simulink model "SimulinkAdsTest"  (R2020b)
(part 2 of 2)

      | 				<Text><![CDATA[InterpolationMode_Previous]]></Text>
      | 				<Enum>1</Enum>
      | 				<Comment><![CDATA[Take previous sample point]]></Comment>
      | 			</EnumInfo>
      | 			<EnumInfo>
      | 				<Text><![CDATA[InterpolationMode_Next]]></Text>
      | 				<Enum>2</Enum>
      | 				<Comment><![CDATA[Take following sample point]]></Comment>
      | 			</EnumInfo>
      | 			<EnumInfo>
      | 				<Text><![CDATA[InterpolationMode_Nearest]]></Text>
      | 				<Enum>3</Enum>
      | 				<Comment><![CDATA[Take nearest sample point]]></Comment>
      | 			</EnumInfo>
      | 			<EnumInfo>
      | 				<Text><![CDATA[InterpolationMode_Linear]]></Text>
      | 				<Enum>4</Enum>
      | 				<Comment><![CDATA[Linear interpolation]]></Comment>
      | 			</EnumInfo>
      | 			<Default>
      | 				<EnumText>InterpolationMode_Nearest</EnumText>
      | 			</Default>
      | 			<Hides>
      | 				<Hide GUID="{D1CE9774-5ABF-42E5-8FE4-99F5DEE76F36}"/>
      | 				<Hide GUID="{430DDA91-6797-4E3C-84C6-A1786F8B6EA7}"/>
      | 				<Hide GUID="{24DF4C47-A5FC-4534-A4AA-304CE11CAE9A}"/>
      | 				<Hide GUID="{5367B9B1-3807-4AFC-B79A-823BBFC694FE}"/>
      | 				<Hide GUID="{36E48A81-1480-4106-A31F-8CC0D9BDE1C1}"/>
      | 				<Hide GUID="{DB809631-0BE7-4AE2-8A30-534C3D3B8C19}"/>
      | 				<Hide GUID="{139A7071-B2F7-4999-AD00-5D72B7A47D1B}"/>
      | 				<Hide GUID="{E828C0A6-3D7C-424C-B6C8-3B4EEF9C18AC}"/>
      | 			</Hides>
      | 		</DataType>
      | 		<DataType>
      | 			<Name GUID="{B2873DF7-0E9A-4371-8FDA-560A407550FC}" Namespace="TcDataExchange">BufferReadExtrapolationMode</Name>
      | 			<BitSize>16</BitSize>
      | 			<BaseType GUID="{18071995-0000-0000-0000-000000000006}">INT</BaseType>
      | 			<EnumInfo>
      | 				<Text><![CDATA[ExtrapolationMode_None]]></Text>
      | 				<Enum>0</Enum>
      | 				<Comment><![CDATA[Return error, if the timestamp is out of the specified range]]></Comment>
      | 			</EnumInfo>
      | 			<EnumInfo>
      | 				<Text><![CDATA[ExtrapolationMode_Constant]]></Text>
      | 				<Enum>1</Enum>
      | 				<Comment><![CDATA[Use nearest sample point, if timestamp is out of the specified range]]></Comment>
      | 			</EnumInfo>
      | 			<EnumInfo>
      | 				<Text><![CDATA[ExtrapolationMode_Linear]]></Text>
      | 				<Enum>2</Enum>
      | 				<Comment><![CDATA[Extrapolate linearly, if timestamp is out of the specified range]]></Comment>
      | 			</EnumInfo>
      | 			<Hides>
      | 				<Hide GUID="{183AB6B0-9D13-4268-9013-6BC144AF43F9}"/>
      | 				<Hide GUID="{58686C98-6145-45BB-A1CE-6DFAFC306DB4}"/>
      | 				<Hide GUID="{EE21BE7C-9D24-4A92-825B-B15B1919983F}"/>
      | 				<Hide GUID="{98B9A1F3-AFB0-4DDD-856E-5CCA2E73CE75}"/>
      | 				<Hide GUID="{34806592-F19E-4DDB-96DC-032ABE8197D4}"/>
      | 				<Hide GUID="{C9391145-9682-4F6A-BF6D-5FA0733C02F4}"/>
      | 				<Hide GUID="{583534AC-9A1B-48FF-99BF-216BF02010E2}"/>
      | 				<Hide GUID="{11A9C8C7-1BFF-45E1-8ABC-29E82EA5F980}"/>
      | 				<Hide GUID="{CA042772-0740-496A-85A1-AE2E06F7EE08}"/>
      | 				<Hide GUID="{7F398EF7-03C7-49DC-B4A8-778E9B813ED0}"/>
      | 				<Hide GUID="{3075835C-D37D-4F7C-8CFA-0A55974D5F50}"/>
      | 			</Hides>
      | 		</DataType>
      | 		<DataType>
      | 			<Name GUID="{D7B34C9A-90C5-4E79-A290-017678319005}" Namespace="TcDataExchange">ITcStreamAdsRequestHandler</Name>
      | 			<BitSize X64="64">32</BitSize>
      | 			<BaseType GUID="{00000001-0000-0000-E000-000000000064}">ITcUnknown</BaseType>
      | 			<Method>
      | 				<Name>Send</Name>
      | 				<ReturnType GUID="{18071995-0000-0000-0000-000000000019}">HRESULT</ReturnType>
      | 				<ReturnBitSize>32</ReturnBitSize>
      | 				<Parameter>
      | 					<Name>timeoutMs</Name>
      | 					<Type GUID="{18071995-0000-0000-0000-000000000006}" Optional="1000">INT</Type>
      | 					<BitSize>16</BitSize>
      | 				</Parameter>
      | 			</Method>
      | 			<Method>
      | 				<Name>GetResult</Name>
      | 				<ReturnType GUID="{18071995-0000-0000-0000-000000000019}">HRESULT</ReturnType>
      | 				<ReturnBitSize>32</ReturnBitSize>
      | 				<Parameter>
      | 					<Name>pErrorCode</Name>
      | 					<Type GUID="{18071995-0000-0000-0000-000000000009}" PointerTo="1" RpcDirection="out">DINT</Type>
      | 					<BitSize X64="64">32</BitSize>
      | 				</Parameter>
      | 				<Parameter>
      | 					<Name>wait</Name>
      | 					<Type GUID="{18071995-0000-0000-0000-000000000030}" Optional="0">BOOL</Type>
      | 					<BitSize>8</BitSize>
      | 				</Parameter>
      | 			</Method>
      | 			<Method>
      | 				<Name>Cancel</Name>
      | 				<ReturnType GUID="{18071995-0000-0000-0000-000000000019}">HRESULT</ReturnType>
      | 				<ReturnBitSize>32</ReturnBitSize>
      | 			</Method>
      | 			<Hides>
      | 				<Hide GUID="{D5D4EABE-5709-4F1D-A52D-DD780CF3BEE8}"/>
      | 				<Hide GUID="{96230612-048D-4927-9A3E-E69B743416F7}"/>
      | 				<Hide GUID="{F0F623C7-A650-457C-A27C-87DC2B08989E}"/>
      | 				<Hide GUID="{18FCA6B6-AFA6-45DD-BC02-F3037EA03FB7}"/>
      | 				<Hide GUID="{12AC5FFF-B3F6-4F3E-8EDD-8044D44F084F}"/>
      | 				<Hide GUID="{6CDF8435-1307-4137-94DE-D793A77839C3}"/>
      | 			</Hides>
      | 		</DataType>
      | 		<DataType>
      | 			<Name GUID="{18071995-0000-0000-0000-000000000041}" TcBaseType="true" HideSubItems="true" CName="AmsNetId">AMSNETID</Name>
      | 			<BitSize>48</BitSize>
      | 			<BaseType GUID="{18071995-0000-0000-0000-000000000001}">BYTE</BaseType>
      | 			<ArrayInfo>
      | 				<LBound>0</LBound>
      | 				<Elements>6</Elements>
      | 			</ArrayInfo>
      | 			<Format>
      | 				<Printf>%d.%d.%d.%d.%d.%d</Printf>
      | 				<Parameter>[0]</Parameter>
      | 				<Parameter>[1]</Parameter>
      | 				<Parameter>[2]</Parameter>
      | 				<Parameter>[3]</Parameter>
      | 				<Parameter>[4]</Parameter>
      | 				<Parameter>[5]</Parameter>
      | 			</Format>
      | 		</DataType>
      | 		<DataType>
      | 			<Name GUID="{18071995-0000-0000-0000-000000000042}" TcBaseType="true" CName="AmsAddr">AMSADDR</Name>
      | 			<BitSize>64</BitSize>
      | 			<SubItem>
      | 				<Name>netId</Name>
      | 				<Type GUID="{18071995-0000-0000-0000-000000000041}">AMSNETID</Type>
      | 				<BitSize>48</BitSize>
      | 				<BitOffs>0</BitOffs>
      | 			</SubItem>
      | 			<SubItem>
      | 				<Name>port</Name>
      | 				<Type GUID="{18071995-0000-0000-0000-000000000004}">WORD</Type>
      | 				<BitSize>16</BitSize>
      | 				<BitOffs>48</BitOffs>
      | 			</SubItem>
      | 			<Format>
      | 				<Printf>%d.%d.%d.%d.%d.%d:%d</Printf>
      | 				<Parameter>.netId[0]</Parameter>
      | 				<Parameter>.netId[1]</Parameter>
      | 				<Parameter>.netId[2]</Parameter>
      | 				<Parameter>.netId[3]</Parameter>
      | 				<Parameter>.netId[4]</Parameter>
      | 				<Parameter>.netId[5]</Parameter>
      | 				<Parameter>.port</Parameter>
      | 			</Format>
      | 			<Format Name="Iec">
      | 				<Printf>(netId:=[%d.%d.%d.%d.%d.%d], port :=%d)</Printf>
      | 				<Parameter>.netId[0]</Parameter>
      | 				<Parameter>.netId[1]</Parameter>
      | 				<Parameter>.netId[2]</Parameter>
      | 				<Parameter>.netId[3]</Parameter>
      | 				<Parameter>.netId[4]</Parameter>
      | 				<Parameter>.netId[5]</Parameter>
      | 				<Parameter>.port</Parameter>
      | 			</Format>
      | 		</DataType>
      | 		<DataType>
      | 			<Name GUID="{2919D6B4-47C4-4AE8-B706-E94C497ECB99}" Namespace="TcDataExchange">NotificationTransMode</Name>
      | 			<BitSize>16</BitSize>
      | 			<BaseType GUID="{18071995-0000-0000-0000-000000000006}">INT</BaseType>
      | 			<EnumInfo>
      | 				<Text><![CDATA[NoTrans]]></Text>
      | 				<Enum>0</Enum>
      | 			</EnumInfo>
      | 			<EnumInfo>
      | 				<Text><![CDATA[ServerCycle]]></Text>
      | 				<Enum>3</Enum>
      | 			</EnumInfo>
      | 			<EnumInfo>
      | 				<Text><![CDATA[OnChange]]></Text>
      | 				<Enum>4</Enum>
      | 			</EnumInfo>
      | 			<Hides>
      | 				<Hide GUID="{79465139-46B4-43EB-B7FF-967BF64C3367}"/>
      | 				<Hide GUID="{AE2F4BB5-B98E-4C79-AC26-086A9CF7EAC6}"/>
      | 				<Hide GUID="{ECF929B2-79C7-483F-A3DC-06B91AFD531C}"/>
      | 				<Hide GUID="{4E4B27B2-E550-42F1-92B6-1EFABDB0481B}"/>
      | 			</Hides>
      | 		</DataType>
      | 		<DataType>
      | 			<Name GUID="{B75DDCED-7BC8-45F5-8D80-27345642612D}" Namespace="TcDataExchange">NotificationState</Name>
      | 			<BitSize>16</BitSize>
      | 			<BaseType GUID="{18071995-0000-0000-0000-000000000006}">INT</BaseType>
      | 			<EnumInfo>
      | 				<Text><![CDATA[Stop]]></Text>
      | 				<Enum>0</Enum>
      | 			</EnumInfo>
      | 			<EnumInfo>
      | 				<Text><![CDATA[Starting]]></Text>
      | 				<Enum>1</Enum>
      | 			</EnumInfo>
      | 			<EnumInfo>
      | 				<Text><![CDATA[Run]]></Text>
      | 				<Enum>2</Enum>
      | 			</EnumInfo>
      | 			<EnumInfo>
      | 				<Text><![CDATA[Stopping]]></Text>
      | 				<Enum>3</Enum>
      | 			</EnumInfo>
      | 			<EnumInfo>
      | 				<Text><![CDATA[StartError]]></Text>
      | 				<Enum>4</Enum>
      | 			</EnumInfo>
      | 			<EnumInfo>
      | 				<Text><![CDATA[StopError]]></Text>
      | 				<Enum>5</Enum>
      | 			</EnumInfo>
      | 			<Hides>
      | 				<Hide GUID="{BEEA3766-C152-4B4D-80E7-6332297C102B}"/>
      | 			</Hides>
      | 		</DataType>
      | 		<DataType>
      | 			<Name GUID="{7BD2CA64-894F-4710-AF21-189254BD7339}" Namespace="TcDataExchange">ITcStreamAdsNotificationHandler</Name>
      | 			<BitSize X64="64">32</BitSize>
      | 			<BaseType GUID="{00000001-0000-0000-E000-000000000064}">ITcUnknown</BaseType>
      | 			<Method>
      | 				<Name>Start</Name>
      | 				<ReturnType GUID="{18071995-0000-0000-0000-000000000019}">HRESULT</ReturnType>
      | 				<ReturnBitSize>32</ReturnBitSize>
      | 				<Parameter>
      | 					<Name>sampleTime100ns</Name>
      | 					<Comment><![CDATA[SampleTime in 100ns. If the value is 0 or too small, the requests will be send as fast as possible.]]></Comment>
      | 					<Type GUID="{18071995-0000-0000-0000-000000000008}" Optional="0">UDINT</Type>
      | 					<BitSize>32</BitSize>
      | 				</Parameter>
      | 				<Parameter>
      | 					<Name>delayTime100ns</Name>
      | 					<Comment><![CDATA[DelayTime in 100ns.]]></Comment>
      | 					<Type GUID="{18071995-0000-0000-0000-000000000008}" Optional="10">UDINT</Type>
      | 					<BitSize>32</BitSize>
      | 				</Parameter>
      | 				<Parameter>
      | 					<Name>createTimeoutMs</Name>
      | 					<Type GUID="{18071995-0000-0000-0000-000000000006}" Optional="1000">INT</Type>
      | 					<BitSize>16</BitSize>
      | 				</Parameter>
      | 				<Parameter>
      | 					<Name>transMode</Name>
      | 					<Type GUID="{2919D6B4-47C4-4AE8-B706-E94C497ECB99}" Namespace="TcDataExchange" Optional="0">NotificationTransMode</Type>
      | 					<BitSize>16</BitSize>
      | 				</Parameter>
      | 			</Method>
      | 			<Method>
      | 				<Name>Stop</Name>
      | 				<ReturnType GUID="{18071995-0000-0000-0000-000000000019}">HRESULT</ReturnType>
      | 				<ReturnBitSize>32</ReturnBitSize>
      | 				<Parameter>
      | 					<Name>stopTimeoutMs</Name>
      | 					<Type GUID="{18071995-0000-0000-0000-000000000006}" Optional="1000">INT</Type>
      | 					<BitSize>16</BitSize>
      | 				</Parameter>
      | 			</Method>
      | 			<Method>
      | 				<Name>GetState</Name>
      | 				<ReturnType GUID="{18071995-0000-0000-0000-000000000019}">HRESULT</ReturnType>
      | 				<ReturnBitSize>32</ReturnBitSize>
      | 				<Parameter>
      | 					<Name>pState</Name>
      | 					<Type GUID="{B75DDCED-7BC8-45F5-8D80-27345642612D}" Namespace="TcDataExchange" PointerTo="1">NotificationState</Type>
      | 					<BitSize X64="64">32</BitSize>
      | 				</Parameter>
      | 				<Parameter>
      | 					<Name>pErrorCode</Name>
      | 					<Type GUID="{18071995-0000-0000-0000-000000000009}" PointerTo="1">DINT</Type>
      | 					<BitSize X64="64">32</BitSize>
      | 				</Parameter>
      | 			</Method>
      | 			<Method>
      | 				<Name>WaitFor</Name>
      | 				<ReturnType GUID="{18071995-0000-0000-0000-000000000019}">HRESULT</ReturnType>
      | 				<ReturnBitSize>32</ReturnBitSize>
      | 				<Parameter>
      | 					<Name>targetState</Name>
      | 					<Type GUID="{B75DDCED-7BC8-45F5-8D80-27345642612D}" Namespace="TcDataExchange">NotificationState</Type>
      | 					<BitSize>16</BitSize>
      | 				</Parameter>
      | 			</Method>
      | 			<Hides>
      | 				<Hide GUID="{0FD54C3A-649C-4819-BA34-40090DB2854F}"/>
      | 				<Hide GUID="{B851627D-4078-4428-873B-9E0DE756697F}"/>
      | 				<Hide GUID="{82738EA0-63AE-4386-9AC8-D5A166BE7CE6}"/>
      | 				<Hide GUID="{62C58600-337E-4913-B519-B241B47A093F}"/>
      | 				<Hide GUID="{F19E62E1-3672-44A5-AE6F-41D70903D13E}"/>
      | 				<Hide GUID="{188DFF90-A46E-4A6C-BF2A-4B79F1A4A7D7}"/>
      | 				<Hide GUID="{20D7666F-EA21-4A02-B0BF-92A2B39D0282}"/>
      | 				<Hide GUID="{B6680295-EE8B-49D4-B982-46287CB9DC7F}"/>
      | 				<Hide GUID="{640F79DB-CF38-45B7-A5A6-1F8ACF6E88C7}"/>
      | 				<Hide GUID="{ACD4E2BC-BCCF-47C3-994A-79C84DA897B4}"/>
      | 			</Hides>
      | 		</DataType>
      | 		<DataType>
      | 			<Name GUID="{44CF19E6-1A23-4E07-B15E-18C86B7D1DF6}" Namespace="TcDataExchange">ITcStreamAdsClient</Name>
      | 			<BitSize X64="64">32</BitSize>
      | 			<BaseType GUID="{00000001-0000-0000-E000-000000000064}">ITcUnknown</BaseType>
      | 			<Method>
      | 				<Name>CreateReadRequest</Name>
      | 				<ReturnType GUID="{18071995-0000-0000-0000-000000000019}">HRESULT</ReturnType>
      | 				<ReturnBitSize>32</ReturnBitSize>
      | 				<Parameter>
      | 					<Name>parentOid</Name>
      | 					<Type GUID="{18071995-0000-0000-0000-00000000000F}">OTCID</Type>
      | 					<BitSize>32</BitSize>
      | 				</Parameter>
      | 				<Parameter>
      | 					<Name>ppRequestHandler</Name>
      | 					<Type GUID="{D7B34C9A-90C5-4E79-A290-017678319005}" Namespace="TcDataExchange" PointerTo="1" RpcDirection="out">ITcStreamAdsRequestHandler</Type>
      | 					<BitSize X64="64">32</BitSize>
      | 				</Parameter>
      | 				<Parameter>
      | 					<Name>amsAddr</Name>
      | 					<Type GUID="{18071995-0000-0000-0000-000000000042}" RpcDirection="in">AMSADDR</Type>
      | 					<BitSize>64</BitSize>
      | 				</Parameter>
      | 				<Parameter>
      | 					<Name>idxGrp</Name>
      | 					<Type GUID="{18071995-0000-0000-0000-000000000008}" RpcDirection="in">UDINT</Type>
      | 					<BitSize>32</BitSize>
      | 				</Parameter>
      | 				<Parameter>
      | 					<Name>idxOffs</Name>
      | 					<Type GUID="{18071995-0000-0000-0000-000000000008}" RpcDirection="in">UDINT</Type>
      | 					<BitSize>32</BitSize>
      | 				</Parameter>
      | 				<Parameter>
      | 					<Name>byteSize</Name>
      | 					<Type GUID="{18071995-0000-0000-0000-000000000008}" RpcDirection="in">UDINT</Type>
      | 					<BitSize>32</BitSize>
      | 				</Parameter>
      | 				<Parameter>
      | 					<Name>pSink</Name>
      | 					<Type GUID="{CD026BE9-DD1E-4238-B09F-CDE426934EFB}" Namespace="TcDataExchange" RpcDirection="in">ITcStreamSyncDataSink</Type>
      | 					<BitSize X64="64">32</BitSize>
      | 				</Parameter>
      | 			</Method>
      | 			<Method>
      | 				<Name>CreateWriteRequest</Name>
      | 				<ReturnType GUID="{18071995-0000-0000-0000-000000000019}">HRESULT</ReturnType>
      | 				<ReturnBitSize>32</ReturnBitSize>
      | 				<Parameter>
      | 					<Name>parentOid</Name>
      | 					<Type GUID="{18071995-0000-0000-0000-00000000000F}">OTCID</Type>
      | 					<BitSize>32</BitSize>
      | 				</Parameter>
      | 				<Parameter>
      | 					<Name>ppRequestHandler</Name>
      | 					<Type GUID="{D7B34C9A-90C5-4E79-A290-017678319005}" Namespace="TcDataExchange" PointerTo="1" RpcDirection="out">ITcStreamAdsRequestHandler</Type>
      | 					<BitSize X64="64">32</BitSize>
      | 				</Parameter>
      | 				<Parameter>
      | 					<Name>amsAddr</Name>
      | 					<Type GUID="{18071995-0000-0000-0000-000000000042}" RpcDirection="in">AMSADDR</Type>
      | 					<BitSize>64</BitSize>
      | 				</Parameter>
      | 				<Parameter>
      | 					<Name>idxGrp</Name>
      | 					<Type GUID="{18071995-0000-0000-0000-000000000008}" RpcDirection="in">UDINT</Type>
      | 					<BitSize>32</BitSize>
      | 				</Parameter>
      | 				<Parameter>
      | 					<Name>idxOffs</Name>
      | 					<Type GUID="{18071995-0000-0000-0000-000000000008}" RpcDirection="in">UDINT</Type>
      | 					<BitSize>32</BitSize>
      | 				</Parameter>
      | 				<Parameter>
      | 					<Name>byteSize</Name>
      | 					<Type GUID="{18071995-0000-0000-0000-000000000008}" RpcDirection="in">UDINT</Type>
      | 					<BitSize>32</BitSize>
      | 				</Parameter>
      | 				<Parameter>
      | 					<Name>pSource</Name>
      | 					<Type GUID="{877CB26F-4EC1-469B-9F87-706DDBDA821F}" Namespace="TcDataExchange" RpcDirection="in">ITcStreamSyncDataSource</Type>
      | 					<BitSize X64="64">32</BitSize>
      | 				</Parameter>
      | 			</Method>
      | 			<Method>
      | 				<Name>CreateReadWriteRequest</Name>
      | 				<ReturnType GUID="{18071995-0000-0000-0000-000000000019}">HRESULT</ReturnType>
      | 				<ReturnBitSize>32</ReturnBitSize>
      | 				<Parameter>
      | 					<Name>parentOid</Name>
      | 					<Type GUID="{18071995-0000-0000-0000-00000000000F}">OTCID</Type>
      | 					<BitSize>32</BitSize>
      | 				</Parameter>
      | 				<Parameter>
      | 					<Name>ppRequestHandler</Name>
      | 					<Type GUID="{D7B34C9A-90C5-4E79-A290-017678319005}" Namespace="TcDataExchange" PointerTo="1" RpcDirection="out">ITcStreamAdsRequestHandler</Type>
      | 					<BitSize X64="64">32</BitSize>
      | 				</Parameter>
      | 				<Parameter>
      | 					<Name>amsAddr</Name>
      | 					<Type GUID="{18071995-0000-0000-0000-000000000042}" RpcDirection="in">AMSADDR</Type>
      | 					<BitSize>64</BitSize>
      | 				</Parameter>
      | 				<Parameter>
      | 					<Name>idxGrp</Name>
      | 					<Type GUID="{18071995-0000-0000-0000-000000000008}" RpcDirection="in">UDINT</Type>
      | 					<BitSize>32</BitSize>
      | 				</Parameter>
      | 				<Parameter>
      | 					<Name>idxOffs</Name>
      | 					<Type GUID="{18071995-0000-0000-0000-000000000008}" RpcDirection="in">UDINT</Type>
      | 					<BitSize>32</BitSize>
      | 				</Parameter>
      | 				<Parameter>
      | 					<Name>writeSize</Name>
      | 					<Type GUID="{18071995-0000-0000-0000-000000000008}" RpcDirection="in">UDINT</Type>
      | 					<BitSize>32</BitSize>
      | 				</Parameter>
      | 				<Parameter>
      | 					<Name>pSource</Name>
      | 					<Type GUID="{877CB26F-4EC1-469B-9F87-706DDBDA821F}" Namespace="TcDataExchange" RpcDirection="in">ITcStreamSyncDataSource</Type>
      | 					<BitSize X64="64">32</BitSize>
      | 				</Parameter>
      | 				<Parameter>
      | 					<Name>readSize</Name>
      | 					<Type GUID="{18071995-0000-0000-0000-000000000008}" RpcDirection="in">UDINT</Type>
      | 					<BitSize>32</BitSize>
      | 				</Parameter>
      | 				<Parameter>
      | 					<Name>pSink</Name>
      | 					<Type GUID="{CD026BE9-DD1E-4238-B09F-CDE426934EFB}" Namespace="TcDataExchange" RpcDirection="in">ITcStreamSyncDataSink</Type>
      | 					<BitSize X64="64">32</BitSize>
      | 				</Parameter>
      | 			</Method>
      | 			<Method>
      | 				<Name>CreateNotificationHandler</Name>
      | 				<ReturnType GUID="{18071995-0000-0000-0000-000000000019}">HRESULT</ReturnType>
      | 				<ReturnBitSize>32</ReturnBitSize>
      | 				<Parameter>
      | 					<Name>parentOid</Name>
      | 					<Type GUID="{18071995-0000-0000-0000-00000000000F}">OTCID</Type>
      | 					<BitSize>32</BitSize>
      | 				</Parameter>
      | 				<Parameter>
      | 					<Name>ppNotificationHandler</Name>
      | 					<Type GUID="{7BD2CA64-894F-4710-AF21-189254BD7339}" Namespace="TcDataExchange" PointerTo="1" RpcDirection="out">ITcStreamAdsNotificationHandler</Type>
      | 					<BitSize X64="64">32</BitSize>
      | 				</Parameter>
      | 				<Parameter>
      | 					<Name>amsAddr</Name>
      | 					<Type GUID="{18071995-0000-0000-0000-000000000042}">AMSADDR</Type>
      | 					<BitSize>64</BitSize>
      | 				</Parameter>
      | 				<Parameter>
      | 					<Name>idxGrp</Name>
      | 					<Type GUID="{18071995-0000-0000-0000-000000000008}" RpcDirection="in">UDINT</Type>
      | 					<BitSize>32</BitSize>
      | 				</Parameter>
      | 				<Parameter>
      | 					<Name>idxOffs</Name>
      | 					<Type GUID="{18071995-0000-0000-0000-000000000008}" RpcDirection="in">UDINT</Type>
      | 					<BitSize>32</BitSize>
      | 				</Parameter>
      | 				<Parameter>
      | 					<Name>byteSize</Name>
      | 					<Type GUID="{18071995-0000-0000-0000-000000000008}" RpcDirection="in">UDINT</Type>
      | 					<BitSize>32</BitSize>
      | 				</Parameter>
      | 				<Parameter>
      | 					<Name>pSink</Name>
      | 					<Type GUID="{CD026BE9-DD1E-4238-B09F-CDE426934EFB}" Namespace="TcDataExchange" RpcDirection="in">ITcStreamSyncDataSink</Type>
      | 					<BitSize X64="64">32</BitSize>
      | 				</Parameter>
      | 			</Method>
      | 			<Hides>
      | 				<Hide GUID="{E5572F78-39F4-4573-890C-3DF0E2006105}"/>
      | 				<Hide GUID="{52252529-8C17-45D1-85B4-6A458C0F3E94}"/>
      | 				<Hide GUID="{F824C7E1-F0C6-44A6-B482-897B83EFF54D}"/>
      | 				<Hide GUID="{89D1DEF9-1EDB-4DC7-B44F-67745448E326}"/>
      | 				<Hide GUID="{9AF2891A-A1C3-41B4-843B-F1318836B90C}"/>
      | 				<Hide GUID="{C92F8EE8-70FC-4938-AE5D-0804054FE778}"/>
      | 				<Hide GUID="{692D2F91-2921-429B-A2FD-B23E2D06FE57}"/>
      | 				<Hide GUID="{247F4AE9-8FC4-4311-BF3B-2963D4FB048A}"/>
      | 				<Hide GUID="{FB8AA9BF-37B4-4992-B5AC-BBA0F4D43373}"/>
      | 				<Hide GUID="{7427C36F-E349-41A6-A066-CB0C042DD556}"/>
      | 				<Hide GUID="{E46C7F48-0073-45AF-850A-7F1CB9D0F1BC}"/>
      | 				<Hide GUID="{096DB961-B576-4662-AA01-00D308385BF0}"/>
      | 				<Hide GUID="{A0AD0C9E-66BD-49F7-B782-910B430A1CD8}"/>
      | 				<Hide GUID="{FA6AC3AF-43AA-44CB-BA36-5723B1AD464D}"/>
      | 				<Hide GUID="{0614F527-21B4-4192-AE03-7FDCC97AD564}"/>
      | 				<Hide GUID="{20F9385A-0313-4208-B227-DA4EACC1424F}"/>
      | 				<Hide GUID="{DBEA0444-99ED-4B99-9B51-31DB70AF46EF}"/>
      | 				<Hide GUID="{C3B2FC5E-7AD1-45D8-9723-AA6C61AD9B60}"/>
      | 				<Hide GUID="{CF97D717-7515-4E5A-BE1F-84F5A676B8F8}"/>
      | 				<Hide GUID="{B3BDED57-1312-4D96-B06F-2628ECBA6EEF}"/>
      | 				<Hide GUID="{5DE91436-84B1-4D76-B0CA-1D6620CA428C}"/>
      | 				<Hide GUID="{A0E457C6-B984-4427-829D-FA992FA6D9F8}"/>
      | 				<Hide GUID="{49669A99-FF7E-4056-9658-FDC96AB6BD99}"/>
      | 				<Hide GUID="{53867E37-5FD2-456B-BE41-4F337E21E47A}"/>
      | 				<Hide GUID="{A3973658-0AF9-4706-9520-0AAF0F575BFE}"/>
      | 				<Hide GUID="{FC062AA8-EE46-46C7-94CF-827603675385}"/>
      | 				<Hide GUID="{021F7DA4-A9B9-4EF5-80F9-A8DBC397B675}"/>
      | 				<Hide GUID="{4D5006B6-E8E6-4498-9498-ACA7E948FC8F}"/>
      | 				<Hide GUID="{984AB404-08AC-4281-AB66-6ED5B3F17DFE}"/>
      | 				<Hide GUID="{D581F6CF-93AC-4E4B-8D6F-3F0EF3492A71}"/>
      | 				<Hide GUID="{7A32D7B0-99BA-4055-815F-11160248ACD0}"/>
      | 				<Hide GUID="{9E7FC559-CAD5-43C8-B16B-2E56C1991573}"/>
      | 				<Hide GUID="{F062CF59-8FAE-4FCB-A01C-9B649900BCA5}"/>
      | 				<Hide GUID="{8728E0D9-0A46-4A30-9F10-DD1BF2EA33CE}"/>
      | 				<Hide GUID="{DFBB006E-343D-4910-A9C8-3AB2FE1535D3}"/>
      | 				<Hide GUID="{28C016BE-C467-4209-83F6-DED24711BF6D}"/>
      | 				<Hide GUID="{090DBC60-C9BC-4AB3-B82F-77F59E060169}"/>
      | 				<Hide GUID="{7C69CB05-063E-4BC5-9379-7224930A2D33}"/>
      | 				<Hide GUID="{AFAD7A5B-01FD-4391-87A6-15283DC78C95}"/>
      | 				<Hide GUID="{5E61A921-550A-4063-9429-A8A28DE5A1E3}"/>
      | 				<Hide GUID="{6BB012C3-FEAE-471E-BD95-27EDA5BB3A24}"/>
      | 				<Hide GUID="{E5B9394C-8543-4D1E-86CA-EC772D80F874}"/>
      | 				<Hide GUID="{B8FC3674-8C27-4962-8D53-5010B3276572}"/>
      | 				<Hide GUID="{7A879166-081C-4396-83F5-1ED6DDC3FE02}"/>
      | 				<Hide GUID="{906345FE-D08D-48EB-B8DC-3909739597CB}"/>
      | 			</Hides>
      | 		</DataType>
      | 	</DataTypes>
      | 	<Translations/>
      | 	<System>
      | 		<Tasks>
      | 			<Task ObjectId="33620000" CycleTime="100000" AmsPort="350" Priority="20">
      | 				<Name>TcDataExchangeModulesTask</Name>
      | 			</Task>
      | 		</Tasks>
      | 		<Modules>
      | 			<Module GUID="{AB7EF359-EC28-4A80-B6B9-1F5FEF806409}" ClassFactoryId="Beckhoff Automation|TcDataExchangeModules|1.0.1.166" Group="DataExchange|StreamUtilities">
      | 				<Name>Synchronizer</Name>
      | 				<CLSID ClassFactory="TcDataExchangeModules">{AB7EF359-EC28-4A80-B6B9-1F5FEF806409}</CLSID>
      | 				<Info/>
      | 				<Licenses>
      | 					<License>
      | 						<LicenseId>{304D006A-8299-4560-AB79-438534B50288}</LicenseId>
      | 					</License>
      | 				</Licenses>
      | 				<InitSequence>SO</InitSequence>
      | 				<Contexts>
      | 					<Context>
      | 						<Id>1</Id>
      | 					</Context>
      | 				</Contexts>
      | 				<Interfaces>
      | 					<Interface DisableCodeGeneration="true">
      | 						<Type GUID="{00000012-0000-0000-E000-000000000064}">ITComObject</Type>
      | 					</Interface>
      | 					<Interface DisableCodeGeneration="true">
      | 						<Type GUID="{03000012-0000-0000-E000-000000000064}">ITcADI</Type>
      | 					</Interface>
      | 					<Interface DisableCodeGeneration="true">
      | 						<Type GUID="{03000018-0000-0000-E000-000000000064}">ITcWatchSource</Type>
      | 					</Interface>
      | 					<Interface>
      | 						<Type GUID="{9165C8A1-78D1-4B81-89D0-BA48F61AF93B}" Namespace="TcDataExchange">ITcStreamSynchronizer</Type>
      | 					</Interface>
      | 				</Interfaces>
      | 				<Parameters>
      | 					<Parameter HideParameter="true">
      | 						<Name>TraceLevelMax</Name>
      | 						<Comment TxtId=""><![CDATA[Controls the amount of log messages.]]></Comment>
      | 						<BitSize>32</BitSize>
      | 						<BaseType GUID="{8007AE3B-86BB-40F2-B385-EF87FCC239A4}">TcTraceLevel</BaseType>
      | 						<PTCID>#x03002103</PTCID>
      | 						<ContextId>1</ContextId>
      | 					</Parameter>
      | 				</Parameters>
      | 				<InstanceName>Synchronizer_Instance1</InstanceName>
      | 				<OTCID>#x01010010</OTCID>
      | 				<ParameterValues>
      | 					<Value>
      | 						<Name>TraceLevelMax</Name>
      | 						<EnumText>tlAlways</EnumText>
      | 					</Value>
      | 				</ParameterValues>
      | 			</Module>
      | 			<Module GUID="{7F2917A9-6092-40A6-BB22-5428D680BA27}" ClassFactoryId="Beckhoff Automation|TcDataExchangeModules|1.0.1.166" Group="DataExchange|StreamUtilities">
      | 				<Name>SyncBuffer</Name>
      | 				<CLSID ClassFactory="TcDataExchangeModules">{7F2917A9-6092-40A6-BB22-5428D680BA27}</CLSID>
      | 				<Info/>
      | 				<Licenses>
      | 					<License>
      | 						<LicenseId>{304D006A-8299-4560-AB79-438534B50288}</LicenseId>
      | 					</License>
      | 				</Licenses>
      | 				<InitSequence>SO</InitSequence>
      | 				<Contexts>
      | 					<Context>
      | 						<Id>1</Id>
      | 					</Context>
      | 				</Contexts>
      | 				<Interfaces>
      | 					<Interface DisableCodeGeneration="true">
      | 						<Type GUID="{00000012-0000-0000-E000-000000000064}">ITComObject</Type>
      | 					</Interface>
      | 					<Interface DisableCodeGeneration="true">
      | 						<Type GUID="{03000012-0000-0000-E000-000000000064}">ITcADI</Type>
      | 					</Interface>
      | 					<Interface DisableCodeGeneration="true">
      | 						<Type GUID="{03000018-0000-0000-E000-000000000064}">ITcWatchSource</Type>
      | 					</Interface>
      | 					<Interface>
      | 						<Type GUID="{CD026BE9-DD1E-4238-B09F-CDE426934EFB}" Namespace="TcDataExchange">ITcStreamSyncDataSink</Type>
      | 					</Interface>
      | 					<Interface>
      | 						<Type GUID="{877CB26F-4EC1-469B-9F87-706DDBDA821F}" Namespace="TcDataExchange">ITcStreamSyncDataSource</Type>
      | 					</Interface>
      | 					<Interface>
      | 						<Type GUID="{CC2323D2-5F91-43AC-9820-54D42A9D0317}" Namespace="TcDataExchange">ITcStreamBuffer</Type>
      | 					</Interface>
      | 				</Interfaces>
      | 				<Parameters>
      | 					<Parameter>
      | 						<Name>InterpolationMode</Name>
      | 						<BitSize>16</BitSize>
      | 						<BaseType GUID="{04A85163-BBE2-45EF-A167-1FD20C2F2D46}" Namespace="TcDataExchange">BufferReadInterpolationMode</BaseType>
      | 						<PTCID>#x00000004</PTCID>
      | 						<ContextId>1</ContextId>
      | 					</Parameter>
      | 					<Parameter>
      | 						<Name>ContinuationMode</Name>
      | 						<BitSize>16</BitSize>
      | 						<BaseType GUID="{B2873DF7-0E9A-4371-8FDA-560A407550FC}" Namespace="TcDataExchange">BufferReadExtrapolationMode</BaseType>
      | 						<PTCID>#x00000005</PTCID>
      | 						<ContextId>1</ContextId>
      | 					</Parameter>
      | 					<Parameter>
      | 						<Name>SampleSize</Name>
      | 						<BitSize>32</BitSize>
      | 						<BaseType GUID="{18071995-0000-0000-0000-000000000008}">UDINT</BaseType>
      | 						<PTCID>#x00000006</PTCID>
      | 						<ContextId>1</ContextId>
      | 					</Parameter>
      | 					<Parameter>
      | 						<Name>Capacity</Name>
      | 						<BitSize>32</BitSize>
      | 						<BaseType GUID="{18071995-0000-0000-0000-000000000008}">UDINT</BaseType>
      | 						<PTCID>#x00000007</PTCID>
      | 						<ContextId>1</ContextId>
      | 					</Parameter>
      | 					<Parameter HideParameter="true">
      | 						<Name>TraceLevelMax</Name>
      | 						<Comment TxtId=""><![CDATA[Controls the amount of log messages.]]></Comment>
      | 						<BitSize>32</BitSize>
      | 						<BaseType GUID="{8007AE3B-86BB-40F2-B385-EF87FCC239A4}">TcTraceLevel</BaseType>
      | 						<PTCID>#x03002103</PTCID>
      | 						<ContextId>1</ContextId>
      | 					</Parameter>
      | 				</Parameters>
      | 				<InterfacePointers>
      | 					<InterfacePointer>
      | 						<PTCID>#x00000001</PTCID>
      | 						<Name>Synchronizer</Name>
      | 						<Type GUID="{9165C8A1-78D1-4B81-89D0-BA48F61AF93B}" Namespace="TcDataExchange">ITcStreamSynchronizer</Type>
      | 						<ContextId>1</ContextId>
      | 					</InterfacePointer>
      | 				</InterfacePointers>
      | 				<InstanceName>SyncBuffer_Instance1</InstanceName>
      | 				<OTCID>#x01010020</OTCID>
      | 				<ParameterValues>
      | 					<Value>
      | 						<Name>InterpolationMode</Name>
      | 						<EnumText>InterpolationMode_Nearest</EnumText>
      | 					</Value>
      | 					<Value>
      | 						<Name>ContinuationMode</Name>
      | 						<EnumText>ExtrapolationMode_None</EnumText>
      | 					</Value>
      | 					<Value>
      | 						<Name>SampleSize</Name>
      | 						<Value>1</Value>
      | 					</Value>
      | 					<Value>
      | 						<Name>Capacity</Name>
      | 						<Value>50</Value>
      | 					</Value>
      | 					<Value>
      | 						<Name>TraceLevelMax</Name>
      | 						<EnumText>tlAlways</EnumText>
      | 					</Value>
      | 				</ParameterValues>
      | 				<InterfacePointerValues>
      | 					<Value>
      | 						<Name>Synchronizer</Name>
      | 						<OTCID>#x01010010</OTCID>
      | 					</Value>
      | 				</InterfacePointerValues>
      | 			</Module>
      | 			<Module GUID="{976B3EC0-C035-4B78-B648-B8952590F899}" ClassFactoryId="Beckhoff Automation|TcDataExchangeModules|1.0.1.166" Group="DataExchange|StreamSinkSource">
      | 				<Name>FromDataArea</Name>
      | 				<CLSID ClassFactory="TcDataExchangeModules">{976B3EC0-C035-4B78-B648-B8952590F899}</CLSID>
      | 				<Info/>
      | 				<Licenses>
      | 					<License>
      | 						<LicenseId>{304D006A-8299-4560-AB79-438534B50288}</LicenseId>
      | 					</License>
      | 				</Licenses>
      | 				<InitSequence>SO</InitSequence>
      | 				<Contexts>
      | 					<Context>
      | 						<Id>1</Id>
      | 					</Context>
      | 				</Contexts>
      | 				<Interfaces>
      | 					<Interface DisableCodeGeneration="true">
      | 						<Type GUID="{00000012-0000-0000-E000-000000000064}">ITComObject</Type>
      | 					</Interface>
      | 					<Interface DisableCodeGeneration="true">
      | 						<Type GUID="{03000012-0000-0000-E000-000000000064}">ITcADI</Type>
      | 					</Interface>
      | 					<Interface DisableCodeGeneration="true">
      | 						<Type GUID="{03000018-0000-0000-E000-000000000064}">ITcWatchSource</Type>
      | 					</Interface>
      | 					<Interface>
      | 						<Type GUID="{03000010-0000-0000-E000-000000000064}">ITcCyclic</Type>
      | 					</Interface>
      | 				</Interfaces>
      | 				<Parameters>
      | 					<Parameter>
      | 						<Name>DataAreaSizes</Name>
      | 						<BitSize>64</BitSize>
      | 						<BaseType GUID="{C636B456-B483-42A5-BD8A-58753433F375}" Namespace="IO">TcIoDataAreaSize</BaseType>
      | 						<PTCID>#x0300002a</PTCID>
      | 						<ContextId>1</ContextId>
      | 					</Parameter>
      | 					<Parameter HideParameter="true">
      | 						<Name>TraceLevelMax</Name>
      | 						<Comment TxtId=""><![CDATA[Controls the amount of log messages.]]></Comment>
      | 						<BitSize>32</BitSize>
      | 						<BaseType GUID="{8007AE3B-86BB-40F2-B385-EF87FCC239A4}">TcTraceLevel</BaseType>
      | 						<PTCID>#x03002103</PTCID>
      | 						<ContextId>1</ContextId>
      | 					</Parameter>
      | 				</Parameters>
      | 				<DataAreas>
      | 					<DataArea DisableCodeGeneration="true">
      | 						<AreaNo AreaType="InputDst" CreateSymbols="true" DynamicArea="true">1</AreaNo>
      | 						<Name>Input</Name>
      | 						<ContextId>1</ContextId>
      | 						<ByteSize>1</ByteSize>
      | 						<Symbol>
      | 							<Name>MAIN.input1</Name>
      | 							<BitSize>8</BitSize>
      | 							<BaseType GUID="{18071995-0000-0000-0000-000000000030}">BOOL</BaseType>
      | 							<PTCID>#x81000000</PTCID>
      | 							<BitOffs>0</BitOffs>
      | 						</Symbol>
      | 					</DataArea>
      | 				</DataAreas>
      | 				<InterfacePointers>
      | 					<InterfacePointer>
      | 						<PTCID>#x00000001</PTCID>
      | 						<Name>DataSink</Name>
      | 						<Type GUID="{CD026BE9-DD1E-4238-B09F-CDE426934EFB}" Namespace="TcDataExchange">ITcStreamSyncDataSink</Type>
      | 						<ContextId>1</ContextId>
      | 					</InterfacePointer>
      | 					<InterfacePointer>
      | 						<PTCID>#x03002060</PTCID>
      | 						<Name>CyclicCaller</Name>
      | 						<Type GUID="{0300001E-0000-0000-E000-000000000064}">ITcCyclicCaller</Type>
      | 						<ContextId>1</ContextId>
      | 					</InterfacePointer>
      | 				</InterfacePointers>
      | 				<InstanceName>FromDataArea_Instance1</InstanceName>
      | 				<OTCID>#x01010030</OTCID>
      | 				<ParameterValues>
      | 					<Value>
      | 						<Name>DataAreaSizes.area</Name>
      | 						<Value>1</Value>
      | 					</Value>
      | 					<Value>
      | 						<Name>DataAreaSizes.size</Name>
      | 						<Value>1</Value>
      | 					</Value>
      | 					<Value>
      | 						<Name>TraceLevelMax</Name>
      | 						<EnumText>tlAlways</EnumText>
      | 					</Value>
      | 				</ParameterValues>
      | 				<InterfacePointerValues>
      | 					<Value>
      | 						<Name>DataSink</Name>
      | 						<OTCID>#x01010020</OTCID>
      | 					</Value>
      | 					<Value>
      | 						<Name>CyclicCaller</Name>
      | 						<OTCID>#x02010020</OTCID>
      | 					</Value>
      | 				</InterfacePointerValues>
      | 			</Module>
      | 			<Module GUID="{E38BFC78-135A-4B90-A7E9-B3ECAB89AD55}" ClassFactoryId="Beckhoff Automation|TcDataExchangeModules|1.0.1.166" Group="DataExchange|Protocols">
      | 				<Name>AdsClient</Name>
      | 				<CLSID ClassFactory="TcDataExchangeModules" RealTimeInstantiable="true">{E38BFC78-135A-4B90-A7E9-B3ECAB89AD55}</CLSID>
      | 				<Info/>
      | 				<Licenses>
      | 					<License>
      | 						<LicenseId>{304D006A-8299-4560-AB79-438534B50288}</LicenseId>
      | 					</License>
      | 				</Licenses>
      | 				<InitSequence>PSO</InitSequence>
      | 				<Contexts>
      | 					<Context>
      | 						<Id>1</Id>
      | 					</Context>
      | 				</Contexts>
      | 				<Interfaces>
      | 					<Interface DisableCodeGeneration="true">
      | 						<Type GUID="{00000012-0000-0000-E000-000000000064}">ITComObject</Type>
      | 					</Interface>
      | 					<Interface DisableCodeGeneration="true">
      | 						<Type GUID="{03000012-0000-0000-E000-000000000064}">ITcADI</Type>
      | 					</Interface>
      | 					<Interface DisableCodeGeneration="true">
      | 						<Type GUID="{03000018-0000-0000-E000-000000000064}">ITcWatchSource</Type>
      | 					</Interface>
      | 					<Interface>
      | 						<Type GUID="{44CF19E6-1A23-4E07-B15E-18C86B7D1DF6}" Namespace="TcDataExchange">ITcStreamAdsClient</Type>
      | 					</Interface>
      | 				</Interfaces>
      | 				<Parameters>
      | 					<Parameter OnlineParameter="true" DisableCodeGeneration="true" ReadOnly="true">
      | 						<Name>LocalNetId</Name>
      | 						<BitSize>48</BitSize>
      | 						<BaseType GUID="{18071995-0000-0000-0000-000000000041}">AMSNETID</BaseType>
      | 						<PTCID>#x00000001</PTCID>
      | 						<ContextId>1</ContextId>
      | 					</Parameter>
      | 					<Parameter>
      | 						<Name>LocalPortNo</Name>
      | 						<BitSize>16</BitSize>
      | 						<BaseType GUID="{18071995-0000-0000-0000-000000000005}">UINT</BaseType>
      | 						<Default>
      | 							<Value>0</Value>
      | 						</Default>
      | 						<PTCID>#x00000002</PTCID>
      | 						<ContextId>1</ContextId>
      | 					</Parameter>
      | 					<Parameter>
      | 						<Name>LocalPortName</Name>
      | 						<BitSize>256</BitSize>
      | 						<BaseType GUID="{18071995-0000-0000-0000-00010000001F}">STRING(31)</BaseType>
      | 						<PTCID>#x00000003</PTCID>
      | 						<ContextId>1</ContextId>
      | 					</Parameter>
      | 					<Parameter HideParameter="true">
      | 						<Name>TraceLevelMax</Name>
      | 						<Comment TxtId=""><![CDATA[Controls the amount of log messages.]]></Comment>
      | 						<BitSize>32</BitSize>
      | 						<BaseType GUID="{8007AE3B-86BB-40F2-B385-EF87FCC239A4}">TcTraceLevel</BaseType>
      | 						<PTCID>#x03002103</PTCID>
      | 						<ContextId>1</ContextId>
      | 					</Parameter>
      | 				</Parameters>
      | 				<InstanceName>AdsClient_Instance1</InstanceName>
      | 				<OTCID>#x01010040</OTCID>
      | 				<ParameterValues>
      | 					<Value>
      | 						<Name>LocalNetId</Name>
      | 						<Data>000000000000</Data>
      | 					</Value>
      | 					<Value>
      | 						<Name>LocalPortNo</Name>
      | 						<Value>0</Value>
      | 					</Value>
      | 					<Value>
      | 						<Name>LocalPortName</Name>
      | 						<String/>
      | 					</Value>
      | 					<Value>
      | 						<Name>TraceLevelMax</Name>
      | 						<EnumText>tlAlways</EnumText>
      | 					</Value>
      | 				</ParameterValues>
      | 			</Module>
      | 			<Module GUID="{2FCAB55D-9E25-4FA5-9A83-9434B5081CA3}" ClassFactoryId="Beckhoff Automation|TcDataExchangeModules|1.0.1.166" Group="DataExchange|StreamSinkSource">
      | 				<Name>FromAndToADS</Name>
      | 				<CLSID ClassFactory="TcDataExchangeModules">{2FCAB55D-9E25-4FA5-9A83-9434B5081CA3}</CLSID>
      | 				<Info/>
      | 				<Licenses>
      | 					<License>
      | 						<LicenseId>{304D006A-8299-4560-AB79-438534B50288}</LicenseId>
      | 					</License>
      | 				</Licenses>
      | 				<InitSequence>SO</InitSequence>
      | 				<Contexts>
      | 					<Context>
      | 						<Id>1</Id>
      | 					</Context>
      | 				</Contexts>
      | 				<Interfaces>
      | 					<Interface DisableCodeGeneration="true">
      | 						<Type GUID="{00000012-0000-0000-E000-000000000064}">ITComObject</Type>
      | 					</Interface>
      | 					<Interface DisableCodeGeneration="true">
      | 						<Type GUID="{03000012-0000-0000-E000-000000000064}">ITcADI</Type>
      | 					</Interface>
      | 					<Interface DisableCodeGeneration="true">
      | 						<Type GUID="{03000018-0000-0000-E000-000000000064}">ITcWatchSource</Type>
      | 					</Interface>
      | 					<Interface>
      | 						<Type GUID="{03000010-0000-0000-E000-000000000064}">ITcCyclic</Type>
      | 					</Interface>
      | 				</Interfaces>
      | 				<Parameters>
      | 					<Parameter>
      | 						<Name>AmsAddr</Name>
      | 						<BitSize>64</BitSize>
      | 						<BaseType GUID="{18071995-0000-0000-0000-000000000042}">AMSADDR</BaseType>
      | 						<PTCID>#x00000005</PTCID>
      | 						<ContextId>1</ContextId>
      | 					</Parameter>
      | 					<Parameter>
      | 						<Name>IndexGroup</Name>
      | 						<BitSize>32</BitSize>
      | 						<BaseType GUID="{18071995-0000-0000-0000-000000000008}">UDINT</BaseType>
      | 						<PTCID>#x00000006</PTCID>
      | 						<ContextId>1</ContextId>
      | 					</Parameter>
      | 					<Parameter>
      | 						<Name>IndexOffset</Name>
      | 						<BitSize>32</BitSize>
      | 						<BaseType GUID="{18071995-0000-0000-0000-000000000008}">UDINT</BaseType>
      | 						<PTCID>#x00000007</PTCID>
      | 						<ContextId>1</ContextId>
      | 					</Parameter>
      | 					<Parameter>
      | 						<Name>ByteSize</Name>
      | 						<BitSize>32</BitSize>
      | 						<BaseType GUID="{18071995-0000-0000-0000-000000000008}">UDINT</BaseType>
      | 						<PTCID>#x00000008</PTCID>
      | 						<ContextId>1</ContextId>
      | 					</Parameter>
      | 					<Parameter>
      | 						<Name>SymbolName</Name>
      | 						<BitSize>2048</BitSize>
      | 						<BaseType GUID="{18071995-0000-0000-0000-0001000000FF}">STRING(255)</BaseType>
      | 						<PTCID>#x00000009</PTCID>
      | 						<ContextId>1</ContextId>
      | 					</Parameter>
      | 					<Parameter>
      | 						<Name>Timeout</Name>
      | 						<BitSize>32</BitSize>
      | 						<BaseType GUID="{18071995-0000-0000-0000-000000000008}">UDINT</BaseType>
      | 						<Unit><![CDATA[ms]]></Unit>
      | 						<Default>
      | 							<Value>1000</Value>
      | 						</Default>
      | 						<PTCID>#x0000000a</PTCID>
      | 						<ContextId>1</ContextId>
      | 					</Parameter>
      | 					<Parameter>
      | 						<Name>ReadViaNotification</Name>
      | 						<BitSize>8</BitSize>
      | 						<BaseType GUID="{18071995-0000-0000-0000-000000000030}">BOOL</BaseType>
      | 						<PTCID>#x0000000b</PTCID>
      | 						<ContextId>1</ContextId>
      | 					</Parameter>
      | 					<Parameter>
      | 						<Name>NotificationTransMode</Name>
      | 						<BitSize>16</BitSize>
      | 						<BaseType GUID="{2919D6B4-47C4-4AE8-B706-E94C497ECB99}" Namespace="TcDataExchange">NotificationTransMode</BaseType>
      | 						<PTCID>#x0000000c</PTCID>
      | 						<ContextId>1</ContextId>
      | 					</Parameter>
      | 					<Parameter>
      | 						<Name>NotificationSampleTime</Name>
      | 						<BitSize>32</BitSize>
      | 						<BaseType GUID="{18071995-0000-0000-0000-000000000008}">UDINT</BaseType>
      | 						<PTCID>#x0000000d</PTCID>
      | 						<ContextId>1</ContextId>
      | 					</Parameter>
      | 					<Parameter>
      | 						<Name>NotificationDelayTime</Name>
      | 						<BitSize>32</BitSize>
      | 						<BaseType GUID="{18071995-0000-0000-0000-000000000008}">UDINT</BaseType>
      | 						<PTCID>#x0000000e</PTCID>
      | 						<ContextId>1</ContextId>
      | 					</Parameter>
      | 					<Parameter HideParameter="true">
      | 						<Name>TraceLevelMax</Name>
      | 						<Comment TxtId=""><![CDATA[Controls the amount of log messages.]]></Comment>
      | 						<BitSize>32</BitSize>
      | 						<BaseType GUID="{8007AE3B-86BB-40F2-B385-EF87FCC239A4}">TcTraceLevel</BaseType>
      | 						<PTCID>#x03002103</PTCID>
      | 						<ContextId>1</ContextId>
      | 					</Parameter>
      | 				</Parameters>
      | 				<InterfacePointers>
      | 					<InterfacePointer>
      | 						<PTCID>#x00000001</PTCID>
      | 						<Name>AdsClient</Name>
      | 						<Type GUID="{44CF19E6-1A23-4E07-B15E-18C86B7D1DF6}" Namespace="TcDataExchange">ITcStreamAdsClient</Type>
      | 						<ContextId>1</ContextId>
      | 					</InterfacePointer>
      | 					<InterfacePointer>
      | 						<PTCID>#x03002060</PTCID>
      | 						<Name>CyclicCaller</Name>
      | 						<Type GUID="{0300001E-0000-0000-E000-000000000064}">ITcCyclicCaller</Type>
      | 						<ContextId>1</ContextId>
      | 					</InterfacePointer>
      | 					<InterfacePointer>
      | 						<PTCID>#x00000003</PTCID>
      | 						<Name>DataSource</Name>
      | 						<Type GUID="{877CB26F-4EC1-469B-9F87-706DDBDA821F}" Namespace="TcDataExchange">ITcStreamSyncDataSource</Type>
      | 						<ContextId>1</ContextId>
      | 					</InterfacePointer>
      | 					<InterfacePointer>
      | 						<PTCID>#x00000004</PTCID>
      | 						<Name>DataSink</Name>
      | 						<Type GUID="{CD026BE9-DD1E-4238-B09F-CDE426934EFB}" Namespace="TcDataExchange">ITcStreamSyncDataSink</Type>
      | 						<ContextId>1</ContextId>
      | 					</InterfacePointer>
      | 				</InterfacePointers>
      | 				<InstanceName>FromAndToADS_Instance1</InstanceName>
      | 				<OTCID>#x01010050</OTCID>
      | 				<ParameterValues>
      | 					<Value>
      | 						<Name>AmsAddr.netId</Name>
      | 						<Data>c0a8089b0101</Data>
      | 					</Value>
      | 					<Value>
      | 						<Name>AmsAddr.port</Name>
      | 						<Value>851</Value>
      | 					</Value>
      | 					<Value>
      | 						<Name>IndexGroup</Name>
      | 						<Value>0</Value>
      | 					</Value>
      | 					<Value>
      | 						<Name>IndexOffset</Name>
      | 						<Value>0</Value>
      | 					</Value>
      | 					<Value>
      | 						<Name>ByteSize</Name>
      | 						<Value>1</Value>
      | 					</Value>
      | 					<Value>
      | 						<Name>SymbolName</Name>
      | 						<String>MAIN.input1</String>
      | 					</Value>
      | 					<Value>
      | 						<Name>Timeout</Name>
      | 						<Value>1000</Value>
      | 					</Value>
      | 					<Value>
      | 						<Name>ReadViaNotification</Name>
      | 						<EnumText>FALSE</EnumText>
      | 					</Value>
      | 					<Value>
      | 						<Name>NotificationTransMode</Name>
      | 						<EnumText>NoTrans</EnumText>
      | 					</Value>
      | 					<Value>
      | 						<Name>NotificationSampleTime</Name>
      | 						<Value>0</Value>
      | 					</Value>
      | 					<Value>
      | 						<Name>NotificationDelayTime</Name>
      | 						<Value>0</Value>
      | 					</Value>
      | 					<Value>
      | 						<Name>TraceLevelMax</Name>
      | 						<EnumText>tlAlways</EnumText>
      | 					</Value>
      | 				</ParameterValues>
      | 				<InterfacePointerValues>
      | 					<Value>
      | 						<Name>AdsClient</Name>
      | 						<OTCID>#x01010040</OTCID>
      | 					</Value>
      | 					<Value>
      | 						<Name>CyclicCaller</Name>
      | 						<OTCID>#x02010020</OTCID>
      | 					</Value>
      | 					<Value>
      | 						<Name>DataSource</Name>
      | 						<OTCID>#x01010020</OTCID>
      | 					</Value>
      | 					<Value>
      | 						<Name>DataSink</Name>
      | 						<OTCID>#x00000000</OTCID>
      | 					</Value>
      | 				</InterfacePointerValues>
      | 			</Module>
      | 			<Module GUID="{7F2917A9-6092-40A6-BB22-5428D680BA27}" ClassFactoryId="Beckhoff Automation|TcDataExchangeModules|1.0.1.166" Group="DataExchange|StreamUtilities">
      | 				<Name>SyncBuffer</Name>
      | 				<CLSID ClassFactory="TcDataExchangeModules">{7F2917A9-6092-40A6-BB22-5428D680BA27}</CLSID>
      | 				<Info/>
      | 				<Licenses>
      | 					<License>
      | 						<LicenseId>{304D006A-8299-4560-AB79-438534B50288}</LicenseId>
      | 					</License>
      | 				</Licenses>
      | 				<InitSequence>SO</InitSequence>
      | 				<Contexts>
      | 					<Context>
      | 						<Id>1</Id>
      | 					</Context>
      | 				</Contexts>
      | 				<Interfaces>
      | 					<Interface DisableCodeGeneration="true">
      | 						<Type GUID="{00000012-0000-0000-E000-000000000064}">ITComObject</Type>
      | 					</Interface>
      | 					<Interface DisableCodeGeneration="true">
      | 						<Type GUID="{03000012-0000-0000-E000-000000000064}">ITcADI</Type>
      | 					</Interface>
      | 					<Interface DisableCodeGeneration="true">
      | 						<Type GUID="{03000018-0000-0000-E000-000000000064}">ITcWatchSource</Type>
      | 					</Interface>
      | 					<Interface>
      | 						<Type GUID="{CD026BE9-DD1E-4238-B09F-CDE426934EFB}" Namespace="TcDataExchange">ITcStreamSyncDataSink</Type>
      | 					</Interface>
      | 					<Interface>
      | 						<Type GUID="{877CB26F-4EC1-469B-9F87-706DDBDA821F}" Namespace="TcDataExchange">ITcStreamSyncDataSource</Type>
      | 					</Interface>
      | 					<Interface>
      | 						<Type GUID="{CC2323D2-5F91-43AC-9820-54D42A9D0317}" Namespace="TcDataExchange">ITcStreamBuffer</Type>
      | 					</Interface>
      | 				</Interfaces>
      | 				<Parameters>
      | 					<Parameter>
      | 						<Name>InterpolationMode</Name>
      | 						<BitSize>16</BitSize>
      | 						<BaseType GUID="{04A85163-BBE2-45EF-A167-1FD20C2F2D46}" Namespace="TcDataExchange">BufferReadInterpolationMode</BaseType>
      | 						<PTCID>#x00000004</PTCID>
      | 						<ContextId>1</ContextId>
      | 					</Parameter>
      | 					<Parameter>
      | 						<Name>ContinuationMode</Name>
      | 						<BitSize>16</BitSize>
      | 						<BaseType GUID="{B2873DF7-0E9A-4371-8FDA-560A407550FC}" Namespace="TcDataExchange">BufferReadExtrapolationMode</BaseType>
      | 						<PTCID>#x00000005</PTCID>
      | 						<ContextId>1</ContextId>
      | 					</Parameter>
      | 					<Parameter>
      | 						<Name>SampleSize</Name>
      | 						<BitSize>32</BitSize>
      | 						<BaseType GUID="{18071995-0000-0000-0000-000000000008}">UDINT</BaseType>
      | 						<PTCID>#x00000006</PTCID>
      | 						<ContextId>1</ContextId>
      | 					</Parameter>
      | 					<Parameter>
      | 						<Name>Capacity</Name>
      | 						<BitSize>32</BitSize>
      | 						<BaseType GUID="{18071995-0000-0000-0000-000000000008}">UDINT</BaseType>
      | 						<PTCID>#x00000007</PTCID>
      | 						<ContextId>1</ContextId>
      | 					</Parameter>
      | 					<Parameter HideParameter="true">
      | 						<Name>TraceLevelMax</Name>
      | 						<Comment TxtId=""><![CDATA[Controls the amount of log messages.]]></Comment>
      | 						<BitSize>32</BitSize>
      | 						<BaseType GUID="{8007AE3B-86BB-40F2-B385-EF87FCC239A4}">TcTraceLevel</BaseType>
      | 						<PTCID>#x03002103</PTCID>
      | 						<ContextId>1</ContextId>
      | 					</Parameter>
      | 				</Parameters>
      | 				<InterfacePointers>
      | 					<InterfacePointer>
      | 						<PTCID>#x00000001</PTCID>
      | 						<Name>Synchronizer</Name>
      | 						<Type GUID="{9165C8A1-78D1-4B81-89D0-BA48F61AF93B}" Namespace="TcDataExchange">ITcStreamSynchronizer</Type>
      | 						<ContextId>1</ContextId>
      | 					</InterfacePointer>
      | 				</InterfacePointers>
      | 				<InstanceName>SyncBuffer_Instance2</InstanceName>
      | 				<OTCID>#x01010060</OTCID>
      | 				<ParameterValues>
      | 					<Value>
      | 						<Name>InterpolationMode</Name>
      | 						<EnumText>InterpolationMode_Nearest</EnumText>
      | 					</Value>
      | 					<Value>
      | 						<Name>ContinuationMode</Name>
      | 						<EnumText>ExtrapolationMode_None</EnumText>
      | 					</Value>
      | 					<Value>
      | 						<Name>SampleSize</Name>
      | 						<Value>1</Value>
      | 					</Value>
      | 					<Value>
      | 						<Name>Capacity</Name>
      | 						<Value>50</Value>
      | 					</Value>
      | 					<Value>
      | 						<Name>TraceLevelMax</Name>
      | 						<EnumText>tlAlways</EnumText>
      | 					</Value>
      | 				</ParameterValues>
      | 				<InterfacePointerValues>
      | 					<Value>
      | 						<Name>Synchronizer</Name>
      | 						<OTCID>#x01010010</OTCID>
      | 					</Value>
      | 				</InterfacePointerValues>
      | 			</Module>
      | 			<Module GUID="{976B3EC0-C035-4B78-B648-B8952590F899}" ClassFactoryId="Beckhoff Automation|TcDataExchangeModules|1.0.1.166" Group="DataExchange|StreamSinkSource">
      | 				<Name>FromDataArea</Name>
      | 				<CLSID ClassFactory="TcDataExchangeModules">{976B3EC0-C035-4B78-B648-B8952590F899}</CLSID>
      | 				<Info/>
      | 				<Licenses>
      | 					<License>
      | 						<LicenseId>{304D006A-8299-4560-AB79-438534B50288}</LicenseId>
      | 					</License>
      | 				</Licenses>
      | 				<InitSequence>SO</InitSequence>
      | 				<Contexts>
      | 					<Context>
      | 						<Id>1</Id>
      | 					</Context>
      | 				</Contexts>
      | 				<Interfaces>
      | 					<Interface DisableCodeGeneration="true">
      | 						<Type GUID="{00000012-0000-0000-E000-000000000064}">ITComObject</Type>
      | 					</Interface>
      | 					<Interface DisableCodeGeneration="true">
      | 						<Type GUID="{03000012-0000-0000-E000-000000000064}">ITcADI</Type>
      | 					</Interface>
      | 					<Interface DisableCodeGeneration="true">
      | 						<Type GUID="{03000018-0000-0000-E000-000000000064}">ITcWatchSource</Type>
      | 					</Interface>
      | 					<Interface>
      | 						<Type GUID="{03000010-0000-0000-E000-000000000064}">ITcCyclic</Type>
      | 					</Interface>
      | 				</Interfaces>
      | 				<Parameters>
      | 					<Parameter>
      | 						<Name>DataAreaSizes</Name>
      | 						<BitSize>64</BitSize>
      | 						<BaseType GUID="{C636B456-B483-42A5-BD8A-58753433F375}" Namespace="IO">TcIoDataAreaSize</BaseType>
      | 						<PTCID>#x0300002a</PTCID>
      | 						<ContextId>1</ContextId>
      | 					</Parameter>
      | 					<Parameter HideParameter="true">
      | 						<Name>TraceLevelMax</Name>
      | 						<Comment TxtId=""><![CDATA[Controls the amount of log messages.]]></Comment>
      | 						<BitSize>32</BitSize>
      | 						<BaseType GUID="{8007AE3B-86BB-40F2-B385-EF87FCC239A4}">TcTraceLevel</BaseType>
      | 						<PTCID>#x03002103</PTCID>
      | 						<ContextId>1</ContextId>
      | 					</Parameter>
      | 				</Parameters>
      | 				<DataAreas>
      | 					<DataArea DisableCodeGeneration="true">
      | 						<AreaNo AreaType="InputDst" CreateSymbols="true" DynamicArea="true">1</AreaNo>
      | 						<Name>Input</Name>
      | 						<ContextId>1</ContextId>
      | 						<ByteSize>1</ByteSize>
      | 						<Symbol>
      | 							<Name>MAIN.input2</Name>
      | 							<BitSize>8</BitSize>
      | 							<BaseType GUID="{18071995-0000-0000-0000-000000000030}">BOOL</BaseType>
      | 							<PTCID>#x81000000</PTCID>
      | 							<BitOffs>0</BitOffs>
      | 						</Symbol>
      | 					</DataArea>
      | 				</DataAreas>
      | 				<InterfacePointers>
      | 					<InterfacePointer>
      | 						<PTCID>#x00000001</PTCID>
      | 						<Name>DataSink</Name>
      | 						<Type GUID="{CD026BE9-DD1E-4238-B09F-CDE426934EFB}" Namespace="TcDataExchange">ITcStreamSyncDataSink</Type>
      | 						<ContextId>1</ContextId>
      | 					</InterfacePointer>
      | 					<InterfacePointer>
      | 						<PTCID>#x03002060</PTCID>
      | 						<Name>CyclicCaller</Name>
      | 						<Type GUID="{0300001E-0000-0000-E000-000000000064}">ITcCyclicCaller</Type>
      | 						<ContextId>1</ContextId>
      | 					</InterfacePointer>
      | 				</InterfacePointers>
      | 				<InstanceName>FromDataArea_Instance2</InstanceName>
      | 				<OTCID>#x01010070</OTCID>
      | 				<ParameterValues>
      | 					<Value>
      | 						<Name>DataAreaSizes.area</Name>
      | 						<Value>1</Value>
      | 					</Value>
      | 					<Value>
      | 						<Name>DataAreaSizes.size</Name>
      | 						<Value>1</Value>
      | 					</Value>
      | 					<Value>
      | 						<Name>TraceLevelMax</Name>
      | 						<EnumText>tlAlways</EnumText>
      | 					</Value>
      | 				</ParameterValues>
      | 				<InterfacePointerValues>
      | 					<Value>
      | 						<Name>DataSink</Name>
      | 						<OTCID>#x01010060</OTCID>
      | 					</Value>
      | 					<Value>
      | 						<Name>CyclicCaller</Name>
      | 						<OTCID>#x02010020</OTCID>
      | 					</Value>
      | 				</InterfacePointerValues>
      | 			</Module>
      | 			<Module GUID="{2FCAB55D-9E25-4FA5-9A83-9434B5081CA3}" ClassFactoryId="Beckhoff Automation|TcDataExchangeModules|1.0.1.166" Group="DataExchange|StreamSinkSource">
      | 				<Name>FromAndToADS</Name>
      | 				<CLSID ClassFactory="TcDataExchangeModules">{2FCAB55D-9E25-4FA5-9A83-9434B5081CA3}</CLSID>
      | 				<Info/>
      | 				<Licenses>
      | 					<License>
      | 						<LicenseId>{304D006A-8299-4560-AB79-438534B50288}</LicenseId>
      | 					</License>
      | 				</Licenses>
      | 				<InitSequence>SO</InitSequence>
      | 				<Contexts>
      | 					<Context>
      | 						<Id>1</Id>
      | 					</Context>
      | 				</Contexts>
      | 				<Interfaces>
      | 					<Interface DisableCodeGeneration="true">
      | 						<Type GUID="{00000012-0000-0000-E000-000000000064}">ITComObject</Type>
      | 					</Interface>
      | 					<Interface DisableCodeGeneration="true">
      | 						<Type GUID="{03000012-0000-0000-E000-000000000064}">ITcADI</Type>
      | 					</Interface>
      | 					<Interface DisableCodeGeneration="true">
      | 						<Type GUID="{03000018-0000-0000-E000-000000000064}">ITcWatchSource</Type>
      | 					</Interface>
      | 					<Interface>
      | 						<Type GUID="{03000010-0000-0000-E000-000000000064}">ITcCyclic</Type>
      | 					</Interface>
      | 				</Interfaces>
      | 				<Parameters>
      | 					<Parameter>
      | 						<Name>AmsAddr</Name>
      | 						<BitSize>64</BitSize>
      | 						<BaseType GUID="{18071995-0000-0000-0000-000000000042}">AMSADDR</BaseType>
      | 						<PTCID>#x00000005</PTCID>
      | 						<ContextId>1</ContextId>
      | 					</Parameter>
      | 					<Parameter>
      | 						<Name>IndexGroup</Name>
      | 						<BitSize>32</BitSize>
      | 						<BaseType GUID="{18071995-0000-0000-0000-000000000008}">UDINT</BaseType>
      | 						<PTCID>#x00000006</PTCID>
      | 						<ContextId>1</ContextId>
      | 					</Parameter>
      | 					<Parameter>
      | 						<Name>IndexOffset</Name>
      | 						<BitSize>32</BitSize>
      | 						<BaseType GUID="{18071995-0000-0000-0000-000000000008}">UDINT</BaseType>
      | 						<PTCID>#x00000007</PTCID>
      | 						<ContextId>1</ContextId>
      | 					</Parameter>
      | 					<Parameter>
      | 						<Name>ByteSize</Name>
      | 						<BitSize>32</BitSize>
      | 						<BaseType GUID="{18071995-0000-0000-0000-000000000008}">UDINT</BaseType>
      | 						<PTCID>#x00000008</PTCID>
      | 						<ContextId>1</ContextId>
      | 					</Parameter>
      | 					<Parameter>
      | 						<Name>SymbolName</Name>
      | 						<BitSize>2048</BitSize>
      | 						<BaseType GUID="{18071995-0000-0000-0000-0001000000FF}">STRING(255)</BaseType>
      | 						<PTCID>#x00000009</PTCID>
      | 						<ContextId>1</ContextId>
      | 					</Parameter>
      | 					<Parameter>
      | 						<Name>Timeout</Name>
      | 						<BitSize>32</BitSize>
      | 						<BaseType GUID="{18071995-0000-0000-0000-000000000008}">UDINT</BaseType>
      | 						<Unit><![CDATA[ms]]></Unit>
      | 						<Default>
      | 							<Value>1000</Value>
      | 						</Default>
      | 						<PTCID>#x0000000a</PTCID>
      | 						<ContextId>1</ContextId>
      | 					</Parameter>
      | 					<Parameter>
      | 						<Name>ReadViaNotification</Name>
      | 						<BitSize>8</BitSize>
      | 						<BaseType GUID="{18071995-0000-0000-0000-000000000030}">BOOL</BaseType>
      | 						<PTCID>#x0000000b</PTCID>
      | 						<ContextId>1</ContextId>
      | 					</Parameter>
      | 					<Parameter>
      | 						<Name>NotificationTransMode</Name>
      | 						<BitSize>16</BitSize>
      | 						<BaseType GUID="{2919D6B4-47C4-4AE8-B706-E94C497ECB99}" Namespace="TcDataExchange">NotificationTransMode</BaseType>
      | 						<PTCID>#x0000000c</PTCID>
      | 						<ContextId>1</ContextId>
      | 					</Parameter>
      | 					<Parameter>
      | 						<Name>NotificationSampleTime</Name>
      | 						<BitSize>32</BitSize>
      | 						<BaseType GUID="{18071995-0000-0000-0000-000000000008}">UDINT</BaseType>
      | 						<PTCID>#x0000000d</PTCID>
      | 						<ContextId>1</ContextId>
      | 					</Parameter>
      | 					<Parameter>
      | 						<Name>NotificationDelayTime</Name>
      | 						<BitSize>32</BitSize>
      | 						<BaseType GUID="{18071995-0000-0000-0000-000000000008}">UDINT</BaseType>
      | 						<PTCID>#x0000000e</PTCID>
      | 						<ContextId>1</ContextId>
      | 					</Parameter>
      | 					<Parameter HideParameter="true">
      | 						<Name>TraceLevelMax</Name>
      | 						<Comment TxtId=""><![CDATA[Controls the amount of log messages.]]></Comment>
      | 						<BitSize>32</BitSize>
      | 						<BaseType GUID="{8007AE3B-86BB-40F2-B385-EF87FCC239A4}">TcTraceLevel</BaseType>
      | 						<PTCID>#x03002103</PTCID>
      | 						<ContextId>1</ContextId>
      | 					</Parameter>
      | 				</Parameters>
      | 				<InterfacePointers>
      | 					<InterfacePointer>
      | 						<PTCID>#x00000001</PTCID>
      | 						<Name>AdsClient</Name>
      | 						<Type GUID="{44CF19E6-1A23-4E07-B15E-18C86B7D1DF6}" Namespace="TcDataExchange">ITcStreamAdsClient</Type>
      | 						<ContextId>1</ContextId>
      | 					</InterfacePointer>
      | 					<InterfacePointer>
      | 						<PTCID>#x03002060</PTCID>
      | 						<Name>CyclicCaller</Name>
      | 						<Type GUID="{0300001E-0000-0000-E000-000000000064}">ITcCyclicCaller</Type>
      | 						<ContextId>1</ContextId>
      | 					</InterfacePointer>
      | 					<InterfacePointer>
      | 						<PTCID>#x00000003</PTCID>
      | 						<Name>DataSource</Name>
      | 						<Type GUID="{877CB26F-4EC1-469B-9F87-706DDBDA821F}" Namespace="TcDataExchange">ITcStreamSyncDataSource</Type>
      | 						<ContextId>1</ContextId>
      | 					</InterfacePointer>
      | 					<InterfacePointer>
      | 						<PTCID>#x00000004</PTCID>
      | 						<Name>DataSink</Name>
      | 						<Type GUID="{CD026BE9-DD1E-4238-B09F-CDE426934EFB}" Namespace="TcDataExchange">ITcStreamSyncDataSink</Type>
      | 						<ContextId>1</ContextId>
      | 					</InterfacePointer>
      | 				</InterfacePointers>
      | 				<InstanceName>FromAndToADS_Instance2</InstanceName>
      | 				<OTCID>#x01010080</OTCID>
      | 				<ParameterValues>
      | 					<Value>
      | 						<Name>AmsAddr.netId</Name>
      | 						<Data>c0a8089b0101</Data>
      | 					</Value>
      | 					<Value>
      | 						<Name>AmsAddr.port</Name>
      | 						<Value>851</Value>
      | 					</Value>
      | 					<Value>
      | 						<Name>IndexGroup</Name>
      | 						<Value>0</Value>
      | 					</Value>
      | 					<Value>
      | 						<Name>IndexOffset</Name>
      | 						<Value>0</Value>
      | 					</Value>
      | 					<Value>
      | 						<Name>ByteSize</Name>
      | 						<Value>1</Value>
      | 					</Value>
      | 					<Value>
      | 						<Name>SymbolName</Name>
      | 						<String>MAIN.input2</String>
      | 					</Value>
      | 					<Value>
      | 						<Name>Timeout</Name>
      | 						<Value>1000</Value>
      | 					</Value>
      | 					<Value>
      | 						<Name>ReadViaNotification</Name>
      | 						<EnumText>FALSE</EnumText>
      | 					</Value>
      | 					<Value>
      | 						<Name>NotificationTransMode</Name>
      | 						<EnumText>NoTrans</EnumText>
      | 					</Value>
      | 					<Value>
      | 						<Name>NotificationSampleTime</Name>
      | 						<Value>0</Value>
      | 					</Value>
      | 					<Value>
      | 						<Name>NotificationDelayTime</Name>
      | 						<Value>0</Value>
      | 					</Value>
      | 					<Value>
      | 						<Name>TraceLevelMax</Name>
      | 						<EnumText>tlAlways</EnumText>
      | 					</Value>
      | 				</ParameterValues>
      | 				<InterfacePointerValues>
      | 					<Value>
      | 						<Name>AdsClient</Name>
      | 						<OTCID>#x01010040</OTCID>
      | 					</Value>
      | 					<Value>
      | 						<Name>CyclicCaller</Name>
      | 						<OTCID>#x02010020</OTCID>
      | 					</Value>
      | 					<Value>
      | 						<Name>DataSource</Name>
      | 						<OTCID>#x01010060</OTCID>
      | 					</Value>
      | 					<Value>
      | 						<Name>DataSink</Name>
      | 						<OTCID>#x00000000</OTCID>
      | 					</Value>
      | 				</InterfacePointerValues>
      | 			</Module>
      | 			<Module GUID="{7F2917A9-6092-40A6-BB22-5428D680BA27}" ClassFactoryId="Beckhoff Automation|TcDataExchangeModules|1.0.1.166" Group="DataExchange|StreamUtilities">
      | 				<Name>SyncBuffer</Name>
      | 				<CLSID ClassFactory="TcDataExchangeModules">{7F2917A9-6092-40A6-BB22-5428D680BA27}</CLSID>
      | 				<Info/>
      | 				<Licenses>
      | 					<License>
      | 						<LicenseId>{304D006A-8299-4560-AB79-438534B50288}</LicenseId>
      | 					</License>
      | 				</Licenses>
      | 				<InitSequence>SO</InitSequence>
      | 				<Contexts>
      | 					<Context>
      | 						<Id>1</Id>
      | 					</Context>
      | 				</Contexts>
      | 				<Interfaces>
      | 					<Interface DisableCodeGeneration="true">
      | 						<Type GUID="{00000012-0000-0000-E000-000000000064}">ITComObject</Type>
      | 					</Interface>
      | 					<Interface DisableCodeGeneration="true">
      | 						<Type GUID="{03000012-0000-0000-E000-000000000064}">ITcADI</Type>
      | 					</Interface>
      | 					<Interface DisableCodeGeneration="true">
      | 						<Type GUID="{03000018-0000-0000-E000-000000000064}">ITcWatchSource</Type>
      | 					</Interface>
      | 					<Interface>
      | 						<Type GUID="{CD026BE9-DD1E-4238-B09F-CDE426934EFB}" Namespace="TcDataExchange">ITcStreamSyncDataSink</Type>
      | 					</Interface>
      | 					<Interface>
      | 						<Type GUID="{877CB26F-4EC1-469B-9F87-706DDBDA821F}" Namespace="TcDataExchange">ITcStreamSyncDataSource</Type>
      | 					</Interface>
      | 					<Interface>
      | 						<Type GUID="{CC2323D2-5F91-43AC-9820-54D42A9D0317}" Namespace="TcDataExchange">ITcStreamBuffer</Type>
      | 					</Interface>
      | 				</Interfaces>
      | 				<Parameters>
      | 					<Parameter>
      | 						<Name>InterpolationMode</Name>
      | 						<BitSize>16</BitSize>
      | 						<BaseType GUID="{04A85163-BBE2-45EF-A167-1FD20C2F2D46}" Namespace="TcDataExchange">BufferReadInterpolationMode</BaseType>
      | 						<PTCID>#x00000004</PTCID>
      | 						<ContextId>1</ContextId>
      | 					</Parameter>
      | 					<Parameter>
      | 						<Name>ContinuationMode</Name>
      | 						<BitSize>16</BitSize>
      | 						<BaseType GUID="{B2873DF7-0E9A-4371-8FDA-560A407550FC}" Namespace="TcDataExchange">BufferReadExtrapolationMode</BaseType>
      | 						<PTCID>#x00000005</PTCID>
      | 						<ContextId>1</ContextId>
      | 					</Parameter>
      | 					<Parameter>
      | 						<Name>SampleSize</Name>
      | 						<BitSize>32</BitSize>
      | 						<BaseType GUID="{18071995-0000-0000-0000-000000000008}">UDINT</BaseType>
      | 						<PTCID>#x00000006</PTCID>
      | 						<ContextId>1</ContextId>
      | 					</Parameter>
      | 					<Parameter>
      | 						<Name>Capacity</Name>
      | 						<BitSize>32</BitSize>
      | 						<BaseType GUID="{18071995-0000-0000-0000-000000000008}">UDINT</BaseType>
      | 						<PTCID>#x00000007</PTCID>
      | 						<ContextId>1</ContextId>
      | 					</Parameter>
      | 					<Parameter HideParameter="true">
      | 						<Name>TraceLevelMax</Name>
      | 						<Comment TxtId=""><![CDATA[Controls the amount of log messages.]]></Comment>
      | 						<BitSize>32</BitSize>
      | 						<BaseType GUID="{8007AE3B-86BB-40F2-B385-EF87FCC239A4}">TcTraceLevel</BaseType>
      | 						<PTCID>#x03002103</PTCID>
      | 						<ContextId>1</ContextId>
      | 					</Parameter>
      | 				</Parameters>
      | 				<InterfacePointers>
      | 					<InterfacePointer>
      | 						<PTCID>#x00000001</PTCID>
      | 						<Name>Synchronizer</Name>
      | 						<Type GUID="{9165C8A1-78D1-4B81-89D0-BA48F61AF93B}" Namespace="TcDataExchange">ITcStreamSynchronizer</Type>
      | 						<ContextId>1</ContextId>
      | 					</InterfacePointer>
      | 				</InterfacePointers>
      | 				<InstanceName>SyncBuffer_Instance3</InstanceName>
      | 				<OTCID>#x01010090</OTCID>
      | 				<ParameterValues>
      | 					<Value>
      | 						<Name>InterpolationMode</Name>
      | 						<EnumText>InterpolationMode_Nearest</EnumText>
      | 					</Value>
      | 					<Value>
      | 						<Name>ContinuationMode</Name>
      | 						<EnumText>ExtrapolationMode_None</EnumText>
      | 					</Value>
      | 					<Value>
      | 						<Name>SampleSize</Name>
      | 						<Value>1</Value>
      | 					</Value>
      | 					<Value>
      | 						<Name>Capacity</Name>
      | 						<Value>50</Value>
      | 					</Value>
      | 					<Value>
      | 						<Name>TraceLevelMax</Name>
      | 						<EnumText>tlAlways</EnumText>
      | 					</Value>
      | 				</ParameterValues>
      | 				<InterfacePointerValues>
      | 					<Value>
      | 						<Name>Synchronizer</Name>
      | 						<OTCID>#x01010010</OTCID>
      | 					</Value>
      | 				</InterfacePointerValues>
      | 			</Module>
      | 			<Module GUID="{976B3EC0-C035-4B78-B648-B8952590F899}" ClassFactoryId="Beckhoff Automation|TcDataExchangeModules|1.0.1.166" Group="DataExchange|StreamSinkSource">
      | 				<Name>FromDataArea</Name>
      | 				<CLSID ClassFactory="TcDataExchangeModules">{976B3EC0-C035-4B78-B648-B8952590F899}</CLSID>
      | 				<Info/>
      | 				<Licenses>
      | 					<License>
      | 						<LicenseId>{304D006A-8299-4560-AB79-438534B50288}</LicenseId>
      | 					</License>
      | 				</Licenses>
      | 				<InitSequence>SO</InitSequence>
      | 				<Contexts>
      | 					<Context>
      | 						<Id>1</Id>
      | 					</Context>
      | 				</Contexts>
      | 				<Interfaces>
      | 					<Interface DisableCodeGeneration="true">
      | 						<Type GUID="{00000012-0000-0000-E000-000000000064}">ITComObject</Type>
      | 					</Interface>
      | 					<Interface DisableCodeGeneration="true">
      | 						<Type GUID="{03000012-0000-0000-E000-000000000064}">ITcADI</Type>
      | 					</Interface>
      | 					<Interface DisableCodeGeneration="true">
      | 						<Type GUID="{03000018-0000-0000-E000-000000000064}">ITcWatchSource</Type>
      | 					</Interface>
      | 					<Interface>
      | 						<Type GUID="{03000010-0000-0000-E000-000000000064}">ITcCyclic</Type>
      | 					</Interface>
      | 				</Interfaces>
      | 				<Parameters>
      | 					<Parameter>
      | 						<Name>DataAreaSizes</Name>
      | 						<BitSize>64</BitSize>
      | 						<BaseType GUID="{C636B456-B483-42A5-BD8A-58753433F375}" Namespace="IO">TcIoDataAreaSize</BaseType>
      | 						<PTCID>#x0300002a</PTCID>
      | 						<ContextId>1</ContextId>
      | 					</Parameter>
      | 					<Parameter HideParameter="true">
      | 						<Name>TraceLevelMax</Name>
      | 						<Comment TxtId=""><![CDATA[Controls the amount of log messages.]]></Comment>
      | 						<BitSize>32</BitSize>
      | 						<BaseType GUID="{8007AE3B-86BB-40F2-B385-EF87FCC239A4}">TcTraceLevel</BaseType>
      | 						<PTCID>#x03002103</PTCID>
      | 						<ContextId>1</ContextId>
      | 					</Parameter>
      | 				</Parameters>
      | 				<DataAreas>
      | 					<DataArea DisableCodeGeneration="true">
      | 						<AreaNo AreaType="InputDst" CreateSymbols="true" DynamicArea="true">1</AreaNo>
      | 						<Name>Input</Name>
      | 						<ContextId>1</ContextId>
      | 						<ByteSize>1</ByteSize>
      | 						<Symbol>
      | 							<Name>MAIN.input3</Name>
      | 							<BitSize>8</BitSize>
      | 							<BaseType GUID="{18071995-0000-0000-0000-000000000030}">BOOL</BaseType>
      | 							<PTCID>#x81000000</PTCID>
      | 							<BitOffs>0</BitOffs>
      | 						</Symbol>
      | 					</DataArea>
      | 				</DataAreas>
      | 				<InterfacePointers>
      | 					<InterfacePointer>
      | 						<PTCID>#x00000001</PTCID>
      | 						<Name>DataSink</Name>
      | 						<Type GUID="{CD026BE9-DD1E-4238-B09F-CDE426934EFB}" Namespace="TcDataExchange">ITcStreamSyncDataSink</Type>
      | 						<ContextId>1</ContextId>
      | 					</InterfacePointer>
      | 					<InterfacePointer>
      | 						<PTCID>#x03002060</PTCID>
      | 						<Name>CyclicCaller</Name>
      | 						<Type GUID="{0300001E-0000-0000-E000-000000000064}">ITcCyclicCaller</Type>
      | 						<ContextId>1</ContextId>
      | 					</InterfacePointer>
      | 				</InterfacePointers>
      | 				<InstanceName>FromDataArea_Instance3</InstanceName>
      | 				<OTCID>#x010100a0</OTCID>
      | 				<ParameterValues>
      | 					<Value>
      | 						<Name>DataAreaSizes.area</Name>
      | 						<Value>1</Value>
      | 					</Value>
      | 					<Value>
      | 						<Name>DataAreaSizes.size</Name>
      | 						<Value>1</Value>
      | 					</Value>
      | 					<Value>
      | 						<Name>TraceLevelMax</Name>
      | 						<EnumText>tlAlways</EnumText>
      | 					</Value>
      | 				</ParameterValues>
      | 				<InterfacePointerValues>
      | 					<Value>
      | 						<Name>DataSink</Name>
      | 						<OTCID>#x01010090</OTCID>
      | 					</Value>
      | 					<Value>
      | 						<Name>CyclicCaller</Name>
      | 						<OTCID>#x02010020</OTCID>
      | 					</Value>
      | 				</InterfacePointerValues>
      | 			</Module>
      | 			<Module GUID="{2FCAB55D-9E25-4FA5-9A83-9434B5081CA3}" ClassFactoryId="Beckhoff Automation|TcDataExchangeModules|1.0.1.166" Group="DataExchange|StreamSinkSource">
      | 				<Name>FromAndToADS</Name>
      | 				<CLSID ClassFactory="TcDataExchangeModules">{2FCAB55D-9E25-4FA5-9A83-9434B5081CA3}</CLSID>
      | 				<Info/>
      | 				<Licenses>
      | 					<License>
      | 						<LicenseId>{304D006A-8299-4560-AB79-438534B50288}</LicenseId>
      | 					</License>
      | 				</Licenses>
      | 				<InitSequence>SO</InitSequence>
      | 				<Contexts>
      | 					<Context>
      | 						<Id>1</Id>
      | 					</Context>
      | 				</Contexts>
      | 				<Interfaces>
      | 					<Interface DisableCodeGeneration="true">
      | 						<Type GUID="{00000012-0000-0000-E000-000000000064}">ITComObject</Type>
      | 					</Interface>
      | 					<Interface DisableCodeGeneration="true">
      | 						<Type GUID="{03000012-0000-0000-E000-000000000064}">ITcADI</Type>
      | 					</Interface>
      | 					<Interface DisableCodeGeneration="true">
      | 						<Type GUID="{03000018-0000-0000-E000-000000000064}">ITcWatchSource</Type>
      | 					</Interface>
      | 					<Interface>
      | 						<Type GUID="{03000010-0000-0000-E000-000000000064}">ITcCyclic</Type>
      | 					</Interface>
      | 				</Interfaces>
      | 				<Parameters>
      | 					<Parameter>
      | 						<Name>AmsAddr</Name>
      | 						<BitSize>64</BitSize>
      | 						<BaseType GUID="{18071995-0000-0000-0000-000000000042}">AMSADDR</BaseType>
      | 						<PTCID>#x00000005</PTCID>
      | 						<ContextId>1</ContextId>
      | 					</Parameter>
      | 					<Parameter>
      | 						<Name>IndexGroup</Name>
      | 						<BitSize>32</BitSize>
      | 						<BaseType GUID="{18071995-0000-0000-0000-000000000008}">UDINT</BaseType>
      | 						<PTCID>#x00000006</PTCID>
      | 						<ContextId>1</ContextId>
      | 					</Parameter>
      | 					<Parameter>
      | 						<Name>IndexOffset</Name>
      | 						<BitSize>32</BitSize>
      | 						<BaseType GUID="{18071995-0000-0000-0000-000000000008}">UDINT</BaseType>
      | 						<PTCID>#x00000007</PTCID>
      | 						<ContextId>1</ContextId>
      | 					</Parameter>
      | 					<Parameter>
      | 						<Name>ByteSize</Name>
      | 						<BitSize>32</BitSize>
      | 						<BaseType GUID="{18071995-0000-0000-0000-000000000008}">UDINT</BaseType>
      | 						<PTCID>#x00000008</PTCID>
      | 						<ContextId>1</ContextId>
      | 					</Parameter>
      | 					<Parameter>
      | 						<Name>SymbolName</Name>
      | 						<BitSize>2048</BitSize>
      | 						<BaseType GUID="{18071995-0000-0000-0000-0001000000FF}">STRING(255)</BaseType>
      | 						<PTCID>#x00000009</PTCID>
      | 						<ContextId>1</ContextId>
      | 					</Parameter>
      | 					<Parameter>
      | 						<Name>Timeout</Name>
      | 						<BitSize>32</BitSize>
      | 						<BaseType GUID="{18071995-0000-0000-0000-000000000008}">UDINT</BaseType>
      | 						<Unit><![CDATA[ms]]></Unit>
      | 						<Default>
      | 							<Value>1000</Value>
      | 						</Default>
      | 						<PTCID>#x0000000a</PTCID>
      | 						<ContextId>1</ContextId>
      | 					</Parameter>
      | 					<Parameter>
      | 						<Name>ReadViaNotification</Name>
      | 						<BitSize>8</BitSize>
      | 						<BaseType GUID="{18071995-0000-0000-0000-000000000030}">BOOL</BaseType>
      | 						<PTCID>#x0000000b</PTCID>
      | 						<ContextId>1</ContextId>
      | 					</Parameter>
      | 					<Parameter>
      | 						<Name>NotificationTransMode</Name>
      | 						<BitSize>16</BitSize>
      | 						<BaseType GUID="{2919D6B4-47C4-4AE8-B706-E94C497ECB99}" Namespace="TcDataExchange">NotificationTransMode</BaseType>
      | 						<PTCID>#x0000000c</PTCID>
      | 						<ContextId>1</ContextId>
      | 					</Parameter>
      | 					<Parameter>
      | 						<Name>NotificationSampleTime</Name>
      | 						<BitSize>32</BitSize>
      | 						<BaseType GUID="{18071995-0000-0000-0000-000000000008}">UDINT</BaseType>
      | 						<PTCID>#x0000000d</PTCID>
      | 						<ContextId>1</ContextId>
      | 					</Parameter>
      | 					<Parameter>
      | 						<Name>NotificationDelayTime</Name>
      | 						<BitSize>32</BitSize>
      | 						<BaseType GUID="{18071995-0000-0000-0000-000000000008}">UDINT</BaseType>
      | 						<PTCID>#x0000000e</PTCID>
      | 						<ContextId>1</ContextId>
      | 					</Parameter>
      | 					<Parameter HideParameter="true">
      | 						<Name>TraceLevelMax</Name>
      | 						<Comment TxtId=""><![CDATA[Controls the amount of log messages.]]></Comment>
      | 						<BitSize>32</BitSize>
      | 						<BaseType GUID="{8007AE3B-86BB-40F2-B385-EF87FCC239A4}">TcTraceLevel</BaseType>
      | 						<PTCID>#x03002103</PTCID>
      | 						<ContextId>1</ContextId>
      | 					</Parameter>
      | 				</Parameters>
      | 				<InterfacePointers>
      | 					<InterfacePointer>
      | 						<PTCID>#x00000001</PTCID>
      | 						<Name>AdsClient</Name>
      | 						<Type GUID="{44CF19E6-1A23-4E07-B15E-18C86B7D1DF6}" Namespace="TcDataExchange">ITcStreamAdsClient</Type>
      | 						<ContextId>1</ContextId>
      | 					</InterfacePointer>
      | 					<InterfacePointer>
      | 						<PTCID>#x03002060</PTCID>
      | 						<Name>CyclicCaller</Name>
      | 						<Type GUID="{0300001E-0000-0000-E000-000000000064}">ITcCyclicCaller</Type>
      | 						<ContextId>1</ContextId>
      | 					</InterfacePointer>
      | 					<InterfacePointer>
      | 						<PTCID>#x00000003</PTCID>
      | 						<Name>DataSource</Name>
      | 						<Type GUID="{877CB26F-4EC1-469B-9F87-706DDBDA821F}" Namespace="TcDataExchange">ITcStreamSyncDataSource</Type>
      | 						<ContextId>1</ContextId>
      | 					</InterfacePointer>
      | 					<InterfacePointer>
      | 						<PTCID>#x00000004</PTCID>
      | 						<Name>DataSink</Name>
      | 						<Type GUID="{CD026BE9-DD1E-4238-B09F-CDE426934EFB}" Namespace="TcDataExchange">ITcStreamSyncDataSink</Type>
      | 						<ContextId>1</ContextId>
      | 					</InterfacePointer>
      | 				</InterfacePointers>
      | 				<InstanceName>FromAndToADS_Instance3</InstanceName>
      | 				<OTCID>#x010100b0</OTCID>
      | 				<ParameterValues>
      | 					<Value>
      | 						<Name>AmsAddr.netId</Name>
      | 						<Data>c0a8089b0101</Data>
      | 					</Value>
      | 					<Value>
      | 						<Name>AmsAddr.port</Name>
      | 						<Value>851</Value>
      | 					</Value>
      | 					<Value>
      | 						<Name>IndexGroup</Name>
      | 						<Value>0</Value>
      | 					</Value>
      | 					<Value>
      | 						<Name>IndexOffset</Name>
      | 						<Value>0</Value>
      | 					</Value>
      | 					<Value>
      | 						<Name>ByteSize</Name>
      | 						<Value>1</Value>
      | 					</Value>
      | 					<Value>
      | 						<Name>SymbolName</Name>
      | 						<String>MAIN.input3</String>
      | 					</Value>
      | 					<Value>
      | 						<Name>Timeout</Name>
      | 						<Value>1000</Value>
      | 					</Value>
      | 					<Value>
      | 						<Name>ReadViaNotification</Name>
      | 						<EnumText>FALSE</EnumText>
      | 					</Value>
      | 					<Value>
      | 						<Name>NotificationTransMode</Name>
      | 						<EnumText>NoTrans</EnumText>
      | 					</Value>
      | 					<Value>
      | 						<Name>NotificationSampleTime</Name>
      | 						<Value>0</Value>
      | 					</Value>
      | 					<Value>
      | 						<Name>NotificationDelayTime</Name>
      | 						<Value>0</Value>
      | 					</Value>
      | 					<Value>
      | 						<Name>TraceLevelMax</Name>
      | 						<EnumText>tlAlways</EnumText>
      | 					</Value>
      | 				</ParameterValues>
      | 				<InterfacePointerValues>
      | 					<Value>
      | 						<Name>AdsClient</Name>
      | 						<OTCID>#x01010040</OTCID>
      | 					</Value>
      | 					<Value>
      | 						<Name>CyclicCaller</Name>
      | 						<OTCID>#x02010020</OTCID>
      | 					</Value>
      | 					<Value>
      | 						<Name>DataSource</Name>
      | 						<OTCID>#x01010090</OTCID>
      | 					</Value>
      | 					<Value>
      | 						<Name>DataSink</Name>
      | 						<OTCID>#x00000000</OTCID>
      | 					</Value>
      | 				</InterfacePointerValues>
      | 			</Module>
      | 			<Module GUID="{7F2917A9-6092-40A6-BB22-5428D680BA27}" ClassFactoryId="Beckhoff Automation|TcDataExchangeModules|1.0.1.166" Group="DataExchange|StreamUtilities">
      | 				<Name>SyncBuffer</Name>
      | 				<CLSID ClassFactory="TcDataExchangeModules">{7F2917A9-6092-40A6-BB22-5428D680BA27}</CLSID>
      | 				<Info/>
      | 				<Licenses>
      | 					<License>
      | 						<LicenseId>{304D006A-8299-4560-AB79-438534B50288}</LicenseId>
      | 					</License>
      | 				</Licenses>
      | 				<InitSequence>SO</InitSequence>
      | 				<Contexts>
      | 					<Context>
      | 						<Id>1</Id>
      | 					</Context>
      | 				</Contexts>
      | 				<Interfaces>
      | 					<Interface DisableCodeGeneration="true">
      | 						<Type GUID="{00000012-0000-0000-E000-000000000064}">ITComObject</Type>
      | 					</Interface>
      | 					<Interface DisableCodeGeneration="true">
      | 						<Type GUID="{03000012-0000-0000-E000-000000000064}">ITcADI</Type>
      | 					</Interface>
      | 					<Interface DisableCodeGeneration="true">
      | 						<Type GUID="{03000018-0000-0000-E000-000000000064}">ITcWatchSource</Type>
      | 					</Interface>
      | 					<Interface>
      | 						<Type GUID="{CD026BE9-DD1E-4238-B09F-CDE426934EFB}" Namespace="TcDataExchange">ITcStreamSyncDataSink</Type>
      | 					</Interface>
      | 					<Interface>
      | 						<Type GUID="{877CB26F-4EC1-469B-9F87-706DDBDA821F}" Namespace="TcDataExchange">ITcStreamSyncDataSource</Type>
      | 					</Interface>
      | 					<Interface>
      | 						<Type GUID="{CC2323D2-5F91-43AC-9820-54D42A9D0317}" Namespace="TcDataExchange">ITcStreamBuffer</Type>
      | 					</Interface>
      | 				</Interfaces>
      | 				<Parameters>
      | 					<Parameter>
      | 						<Name>InterpolationMode</Name>
      | 						<BitSize>16</BitSize>
      | 						<BaseType GUID="{04A85163-BBE2-45EF-A167-1FD20C2F2D46}" Namespace="TcDataExchange">BufferReadInterpolationMode</BaseType>
      | 						<PTCID>#x00000004</PTCID>
      | 						<ContextId>1</ContextId>
      | 					</Parameter>
      | 					<Parameter>
      | 						<Name>ContinuationMode</Name>
      | 						<BitSize>16</BitSize>
      | 						<BaseType GUID="{B2873DF7-0E9A-4371-8FDA-560A407550FC}" Namespace="TcDataExchange">BufferReadExtrapolationMode</BaseType>
      | 						<PTCID>#x00000005</PTCID>
      | 						<ContextId>1</ContextId>
      | 					</Parameter>
      | 					<Parameter>
      | 						<Name>SampleSize</Name>
      | 						<BitSize>32</BitSize>
      | 						<BaseType GUID="{18071995-0000-0000-0000-000000000008}">UDINT</BaseType>
      | 						<PTCID>#x00000006</PTCID>
      | 						<ContextId>1</ContextId>
      | 					</Parameter>
      | 					<Parameter>
      | 						<Name>Capacity</Name>
      | 						<BitSize>32</BitSize>
      | 						<BaseType GUID="{18071995-0000-0000-0000-000000000008}">UDINT</BaseType>
      | 						<PTCID>#x00000007</PTCID>
      | 						<ContextId>1</ContextId>
      | 					</Parameter>
      | 					<Parameter HideParameter="true">
      | 						<Name>TraceLevelMax</Name>
      | 						<Comment TxtId=""><![CDATA[Controls the amount of log messages.]]></Comment>
      | 						<BitSize>32</BitSize>
      | 						<BaseType GUID="{8007AE3B-86BB-40F2-B385-EF87FCC239A4}">TcTraceLevel</BaseType>
      | 						<PTCID>#x03002103</PTCID>
      | 						<ContextId>1</ContextId>
      | 					</Parameter>
      | 				</Parameters>
      | 				<InterfacePointers>
      | 					<InterfacePointer>
      | 						<PTCID>#x00000001</PTCID>
      | 						<Name>Synchronizer</Name>
      | 						<Type GUID="{9165C8A1-78D1-4B81-89D0-BA48F61AF93B}" Namespace="TcDataExchange">ITcStreamSynchronizer</Type>
      | 						<ContextId>1</ContextId>
      | 					</InterfacePointer>
      | 				</InterfacePointers>
      | 				<InstanceName>SyncBuffer_Instance4</InstanceName>
      | 				<OTCID>#x010100c0</OTCID>
      | 				<ParameterValues>
      | 					<Value>
      | 						<Name>InterpolationMode</Name>
      | 						<EnumText>InterpolationMode_Nearest</EnumText>
      | 					</Value>
      | 					<Value>
      | 						<Name>ContinuationMode</Name>
      | 						<EnumText>ExtrapolationMode_None</EnumText>
      | 					</Value>
      | 					<Value>
      | 						<Name>SampleSize</Name>
      | 						<Value>1</Value>
      | 					</Value>
      | 					<Value>
      | 						<Name>Capacity</Name>
      | 						<Value>50</Value>
      | 					</Value>
      | 					<Value>
      | 						<Name>TraceLevelMax</Name>
      | 						<EnumText>tlAlways</EnumText>
      | 					</Value>
      | 				</ParameterValues>
      | 				<InterfacePointerValues>
      | 					<Value>
      | 						<Name>Synchronizer</Name>
      | 						<OTCID>#x01010010</OTCID>
      | 					</Value>
      | 				</InterfacePointerValues>
      | 			</Module>
      | 			<Module GUID="{2FCAB55D-9E25-4FA5-9A83-9434B5081CA3}" ClassFactoryId="Beckhoff Automation|TcDataExchangeModules|1.0.1.166" Group="DataExchange|StreamSinkSource">
      | 				<Name>FromAndToADS</Name>
      | 				<CLSID ClassFactory="TcDataExchangeModules">{2FCAB55D-9E25-4FA5-9A83-9434B5081CA3}</CLSID>
      | 				<Info/>
      | 				<Licenses>
      | 					<License>
      | 						<LicenseId>{304D006A-8299-4560-AB79-438534B50288}</LicenseId>
      | 					</License>
      | 				</Licenses>
      | 				<InitSequence>SO</InitSequence>
      | 				<Contexts>
      | 					<Context>
      | 						<Id>1</Id>
      | 					</Context>
      | 				</Contexts>
      | 				<Interfaces>
      | 					<Interface DisableCodeGeneration="true">
      | 						<Type GUID="{00000012-0000-0000-E000-000000000064}">ITComObject</Type>
      | 					</Interface>
      | 					<Interface DisableCodeGeneration="true">
      | 						<Type GUID="{03000012-0000-0000-E000-000000000064}">ITcADI</Type>
      | 					</Interface>
      | 					<Interface DisableCodeGeneration="true">
      | 						<Type GUID="{03000018-0000-0000-E000-000000000064}">ITcWatchSource</Type>
      | 					</Interface>
      | 					<Interface>
      | 						<Type GUID="{03000010-0000-0000-E000-000000000064}">ITcCyclic</Type>
      | 					</Interface>
      | 				</Interfaces>
      | 				<Parameters>
      | 					<Parameter>
      | 						<Name>AmsAddr</Name>
      | 						<BitSize>64</BitSize>
      | 						<BaseType GUID="{18071995-0000-0000-0000-000000000042}">AMSADDR</BaseType>
      | 						<PTCID>#x00000005</PTCID>
      | 						<ContextId>1</ContextId>
      | 					</Parameter>
      | 					<Parameter>
      | 						<Name>IndexGroup</Name>
      | 						<BitSize>32</BitSize>
      | 						<BaseType GUID="{18071995-0000-0000-0000-000000000008}">UDINT</BaseType>
      | 						<PTCID>#x00000006</PTCID>
      | 						<ContextId>1</ContextId>
      | 					</Parameter>
      | 					<Parameter>
      | 						<Name>IndexOffset</Name>
      | 						<BitSize>32</BitSize>
      | 						<BaseType GUID="{18071995-0000-0000-0000-000000000008}">UDINT</BaseType>
      | 						<PTCID>#x00000007</PTCID>
      | 						<ContextId>1</ContextId>
      | 					</Parameter>
      | 					<Parameter>
      | 						<Name>ByteSize</Name>
      | 						<BitSize>32</BitSize>
      | 						<BaseType GUID="{18071995-0000-0000-0000-000000000008}">UDINT</BaseType>
      | 						<PTCID>#x00000008</PTCID>
      | 						<ContextId>1</ContextId>
      | 					</Parameter>
      | 					<Parameter>
      | 						<Name>SymbolName</Name>
      | 						<BitSize>2048</BitSize>
      | 						<BaseType GUID="{18071995-0000-0000-0000-0001000000FF}">STRING(255)</BaseType>
      | 						<PTCID>#x00000009</PTCID>
      | 						<ContextId>1</ContextId>
      | 					</Parameter>
      | 					<Parameter>
      | 						<Name>Timeout</Name>
      | 						<BitSize>32</BitSize>
      | 						<BaseType GUID="{18071995-0000-0000-0000-000000000008}">UDINT</BaseType>
      | 						<Unit><![CDATA[ms]]></Unit>
      | 						<Default>
      | 							<Value>1000</Value>
      | 						</Default>
      | 						<PTCID>#x0000000a</PTCID>
      | 						<ContextId>1</ContextId>
      | 					</Parameter>
      | 					<Parameter>
      | 						<Name>ReadViaNotification</Name>
      | 						<BitSize>8</BitSize>
      | 						<BaseType GUID="{18071995-0000-0000-0000-000000000030}">BOOL</BaseType>
      | 						<PTCID>#x0000000b</PTCID>
      | 						<ContextId>1</ContextId>
      | 					</Parameter>
      | 					<Parameter>
      | 						<Name>NotificationTransMode</Name>
      | 						<BitSize>16</BitSize>
      | 						<BaseType GUID="{2919D6B4-47C4-4AE8-B706-E94C497ECB99}" Namespace="TcDataExchange">NotificationTransMode</BaseType>
      | 						<PTCID>#x0000000c</PTCID>
      | 						<ContextId>1</ContextId>
      | 					</Parameter>
      | 					<Parameter>
      | 						<Name>NotificationSampleTime</Name>
      | 						<BitSize>32</BitSize>
      | 						<BaseType GUID="{18071995-0000-0000-0000-000000000008}">UDINT</BaseType>
      | 						<PTCID>#x0000000d</PTCID>
      | 						<ContextId>1</ContextId>
      | 					</Parameter>
      | 					<Parameter>
      | 						<Name>NotificationDelayTime</Name>
      | 						<BitSize>32</BitSize>
      | 						<BaseType GUID="{18071995-0000-0000-0000-000000000008}">UDINT</BaseType>
      | 						<PTCID>#x0000000e</PTCID>
      | 						<ContextId>1</ContextId>
      | 					</Parameter>
      | 					<Parameter HideParameter="true">
      | 						<Name>TraceLevelMax</Name>
      | 						<Comment TxtId=""><![CDATA[Controls the amount of log messages.]]></Comment>
      | 						<BitSize>32</BitSize>
      | 						<BaseType GUID="{8007AE3B-86BB-40F2-B385-EF87FCC239A4}">TcTraceLevel</BaseType>
      | 						<PTCID>#x03002103</PTCID>
      | 						<ContextId>1</ContextId>
      | 					</Parameter>
      | 				</Parameters>
      | 				<InterfacePointers>
      | 					<InterfacePointer>
      | 						<PTCID>#x00000001</PTCID>
      | 						<Name>AdsClient</Name>
      | 						<Type GUID="{44CF19E6-1A23-4E07-B15E-18C86B7D1DF6}" Namespace="TcDataExchange">ITcStreamAdsClient</Type>
      | 						<ContextId>1</ContextId>
      | 					</InterfacePointer>
      | 					<InterfacePointer>
      | 						<PTCID>#x03002060</PTCID>
      | 						<Name>CyclicCaller</Name>
      | 						<Type GUID="{0300001E-0000-0000-E000-000000000064}">ITcCyclicCaller</Type>
      | 						<ContextId>1</ContextId>
      | 					</InterfacePointer>
      | 					<InterfacePointer>
      | 						<PTCID>#x00000003</PTCID>
      | 						<Name>DataSource</Name>
      | 						<Type GUID="{877CB26F-4EC1-469B-9F87-706DDBDA821F}" Namespace="TcDataExchange">ITcStreamSyncDataSource</Type>
      | 						<ContextId>1</ContextId>
      | 					</InterfacePointer>
      | 					<InterfacePointer>
      | 						<PTCID>#x00000004</PTCID>
      | 						<Name>DataSink</Name>
      | 						<Type GUID="{CD026BE9-DD1E-4238-B09F-CDE426934EFB}" Namespace="TcDataExchange">ITcStreamSyncDataSink</Type>
      | 						<ContextId>1</ContextId>
      | 					</InterfacePointer>
      | 				</InterfacePointers>
      | 				<InstanceName>FromAndToADS_Instance4</InstanceName>
      | 				<OTCID>#x010100d0</OTCID>
      | 				<ParameterValues>
      | 					<Value>
      | 						<Name>AmsAddr.netId</Name>
      | 						<Data>c0a8089b0101</Data>
      | 					</Value>
      | 					<Value>
      | 						<Name>AmsAddr.port</Name>
      | 						<Value>851</Value>
      | 					</Value>
      | 					<Value>
      | 						<Name>IndexGroup</Name>
      | 						<Value>0</Value>
      | 					</Value>
      | 					<Value>
      | 						<Name>IndexOffset</Name>
      | 						<Value>0</Value>
      | 					</Value>
      | 					<Value>
      | 						<Name>ByteSize</Name>
      | 						<Value>1</Value>
      | 					</Value>
      | 					<Value>
      | 						<Name>SymbolName</Name>
      | 						<String>MAIN.SchieberOben</String>
      | 					</Value>
      | 					<Value>
      | 						<Name>Timeout</Name>
      | 						<Value>1000</Value>
      | 					</Value>
      | 					<Value>
      | 						<Name>ReadViaNotification</Name>
      | 						<EnumText>TRUE</EnumText>
      | 					</Value>
      | 					<Value>
      | 						<Name>NotificationTransMode</Name>
      | 						<EnumText>ServerCycle</EnumText>
      | 					</Value>
      | 					<Value>
      | 						<Name>NotificationSampleTime</Name>
      | 						<Value>100000</Value>
      | 					</Value>
      | 					<Value>
      | 						<Name>NotificationDelayTime</Name>
      | 						<Value>1000000</Value>
      | 					</Value>
      | 					<Value>
      | 						<Name>TraceLevelMax</Name>
      | 						<EnumText>tlAlways</EnumText>
      | 					</Value>
      | 				</ParameterValues>
      | 				<InterfacePointerValues>
      | 					<Value>
      | 						<Name>AdsClient</Name>
      | 						<OTCID>#x01010040</OTCID>
      | 					</Value>
      | 					<Value>
      | 						<Name>CyclicCaller</Name>
      | 						<OTCID>#x02010020</OTCID>
      | 					</Value>
      | 					<Value>
      | 						<Name>DataSource</Name>
      | 						<OTCID>#x00000000</OTCID>
      | 					</Value>
      | 					<Value>
      | 						<Name>DataSink</Name>
      | 						<OTCID>#x010100c0</OTCID>
      | 					</Value>
      | 				</InterfacePointerValues>
      | 			</Module>
      | 			<Module GUID="{0D48E1A1-2F46-4184-A85B-04744F5D3239}" ClassFactoryId="Beckhoff Automation|TcDataExchangeModules|1.0.1.166" Group="DataExchange|StreamSinkSource">
      | 				<Name>ToDataArea</Name>
      | 				<CLSID ClassFactory="TcDataExchangeModules">{0D48E1A1-2F46-4184-A85B-04744F5D3239}</CLSID>
      | 				<Info/>
      | 				<Licenses>
      | 					<License>
      | 						<LicenseId>{304D006A-8299-4560-AB79-438534B50288}</LicenseId>
      | 					</License>
      | 				</Licenses>
      | 				<InitSequence>SO</InitSequence>
      | 				<Contexts>
      | 					<Context>
      | 						<Id>1</Id>
      | 					</Context>
      | 				</Contexts>
      | 				<Interfaces>
      | 					<Interface DisableCodeGeneration="true">
      | 						<Type GUID="{00000012-0000-0000-E000-000000000064}">ITComObject</Type>
      | 					</Interface>
      | 					<Interface DisableCodeGeneration="true">
      | 						<Type GUID="{03000012-0000-0000-E000-000000000064}">ITcADI</Type>
      | 					</Interface>
      | 					<Interface DisableCodeGeneration="true">
      | 						<Type GUID="{03000018-0000-0000-E000-000000000064}">ITcWatchSource</Type>
      | 					</Interface>
      | 					<Interface>
      | 						<Type GUID="{03000010-0000-0000-E000-000000000064}">ITcCyclic</Type>
      | 					</Interface>
      | 				</Interfaces>
      | 				<Parameters>
      | 					<Parameter>
      | 						<Name>DataAreaSizes</Name>
      | 						<BitSize>64</BitSize>
      | 						<BaseType GUID="{C636B456-B483-42A5-BD8A-58753433F375}" Namespace="IO">TcIoDataAreaSize</BaseType>
      | 						<PTCID>#x0300002a</PTCID>
      | 						<ContextId>1</ContextId>
      | 					</Parameter>
      | 					<Parameter HideParameter="true">
      | 						<Name>TraceLevelMax</Name>
      | 						<Comment TxtId=""><![CDATA[Controls the amount of log messages.]]></Comment>
      | 						<BitSize>32</BitSize>
      | 						<BaseType GUID="{8007AE3B-86BB-40F2-B385-EF87FCC239A4}">TcTraceLevel</BaseType>
      | 						<PTCID>#x03002103</PTCID>
      | 						<ContextId>1</ContextId>
      | 					</Parameter>
      | 				</Parameters>
      | 				<DataAreas>
      | 					<DataArea DisableCodeGeneration="true">
      | 						<AreaNo AreaType="OutputSrc" CreateSymbols="true" DynamicArea="true">1</AreaNo>
      | 						<Name>Output</Name>
      | 						<ContextId>1</ContextId>
      | 						<ByteSize>1</ByteSize>
      | 						<Symbol>
      | 							<Name>MAIN.SchieberOben</Name>
      | 							<BitSize>8</BitSize>
      | 							<BaseType GUID="{18071995-0000-0000-0000-000000000030}">BOOL</BaseType>
      | 							<PTCID>#x81000000</PTCID>
      | 							<BitOffs>0</BitOffs>
      | 						</Symbol>
      | 					</DataArea>
      | 				</DataAreas>
      | 				<InterfacePointers>
      | 					<InterfacePointer>
      | 						<PTCID>#x00000001</PTCID>
      | 						<Name>DataSource</Name>
      | 						<Type GUID="{877CB26F-4EC1-469B-9F87-706DDBDA821F}" Namespace="TcDataExchange">ITcStreamSyncDataSource</Type>
      | 						<ContextId>1</ContextId>
      | 					</InterfacePointer>
      | 					<InterfacePointer>
      | 						<PTCID>#x03002060</PTCID>
      | 						<Name>CyclicCaller</Name>
      | 						<Type GUID="{0300001E-0000-0000-E000-000000000064}">ITcCyclicCaller</Type>
      | 						<ContextId>1</ContextId>
      | 					</InterfacePointer>
      | 				</InterfacePointers>
      | 				<InstanceName>ToDataArea_Instance1</InstanceName>
      | 				<OTCID>#x010100e0</OTCID>
      | 				<ParameterValues>
      | 					<Value>
      | 						<Name>DataAreaSizes.area</Name>
      | 						<Value>1</Value>
      | 					</Value>
      | 					<Value>
      | 						<Name>DataAreaSizes.size</Name>
      | 						<Value>1</Value>
      | 					</Value>
      | 					<Value>
      | 						<Name>TraceLevelMax</Name>
      | 						<EnumText>tlAlways</EnumText>
      | 					</Value>
      | 				</ParameterValues>
      | 				<InterfacePointerValues>
      | 					<Value>
      | 						<Name>DataSource</Name>
      | 						<OTCID>#x010100c0</OTCID>
      | 					</Value>
      | 					<Value>
      | 						<Name>CyclicCaller</Name>
      | 						<OTCID>#x02010020</OTCID>
      | 					</Value>
      | 				</InterfacePointerValues>
      | 			</Module>
      | 		</Modules>
      | 	</System>
      | </TcRuntimAdapterProject>
      | <PortInfo>
      | 	<Inputs>
      | 		<SymbolControlItems>
      | 			<SymbolControlItem GroupName="ADS Write" GroupDescription="Parameters for ADS Write command">
      | 				<Parameters>
      | 					<Parameter Name="Name">MAIN.input1</Parameter>
      | 					<Parameter Name="SymbolName">MAIN.input1</Parameter>
      | 					<Parameter Name="SymbolType">BOOL</Parameter>
      | 					<Parameter Name="SymbolGuid">{18071995-0000-0000-0000-000000000030}</Parameter>
      | 					<Parameter Name="AmsNetId">192.168.8.155.1.1</Parameter>
      | 					<Parameter Name="Port">851</Parameter>
      | 					<Parameter Name="IndexGroup">#x0</Parameter>
      | 					<Parameter Name="IndexOffset">#x0</Parameter>
      | 					<Parameter Name="BitSize">8</Parameter>
      | 					<Parameter Name="InterpolationMode">3</Parameter>
      | 					<Parameter Name="ExtrapolationMode">0</Parameter>
      | 					<Parameter Name="SampleTime TC[100ns]">100000</Parameter>
      | 					<Parameter Name="SampleTime">100000</Parameter>
      | 					<Parameter Name="Timeout">1000</Parameter>
      | 					<Parameter Name="BufferSize">50</Parameter>
      | 				</Parameters>
      | 			</SymbolControlItem>
      | 			<SymbolControlItem GroupName="ADS Write" GroupDescription="Parameters for ADS Write command">
      | 				<Parameters>
      | 					<Parameter Name="Name">MAIN.input2</Parameter>
      | 					<Parameter Name="SymbolName">MAIN.input2</Parameter>
      | 					<Parameter Name="SymbolType">BOOL</Parameter>
      | 					<Parameter Name="SymbolGuid">{18071995-0000-0000-0000-000000000030}</Parameter>
      | 					<Parameter Name="AmsNetId">192.168.8.155.1.1</Parameter>
      | 					<Parameter Name="Port">851</Parameter>
      | 					<Parameter Name="IndexGroup">#x0</Parameter>
      | 					<Parameter Name="IndexOffset">#x0</Parameter>
      | 					<Parameter Name="BitSize">8</Parameter>
      | 					<Parameter Name="InterpolationMode">3</Parameter>
      | 					<Parameter Name="ExtrapolationMode">0</Parameter>
      | 					<Parameter Name="SampleTime TC[100ns]">100000</Parameter>
      | 					<Parameter Name="SampleTime">100000</Parameter>
      | 					<Parameter Name="Timeout">1000</Parameter>
      | 					<Parameter Name="BufferSize">50</Parameter>
      | 				</Parameters>
      | 			</SymbolControlItem>
      | 			<SymbolControlItem GroupName="ADS Write" GroupDescription="Parameters for ADS Write command">
      | 				<Parameters>
      | 					<Parameter Name="Name">MAIN.input3</Parameter>
      | 					<Parameter Name="SymbolName">MAIN.input3</Parameter>
      | 					<Parameter Name="SymbolType">BOOL</Parameter>
      | 					<Parameter Name="SymbolGuid">{18071995-0000-0000-0000-000000000030}</Parameter>
      | 					<Parameter Name="AmsNetId">192.168.8.155.1.1</Parameter>
      | 					<Parameter Name="Port">851</Parameter>
      | 					<Parameter Name="IndexGroup">#x0</Parameter>
      | 					<Parameter Name="IndexOffset">#x0</Parameter>
      | 					<Parameter Name="BitSize">8</Parameter>
      | 					<Parameter Name="InterpolationMode">3</Parameter>
      | 					<Parameter Name="ExtrapolationMode">0</Parameter>
      | 					<Parameter Name="SampleTime TC[100ns]">100000</Parameter>
      | 					<Parameter Name="SampleTime">100000</Parameter>
      | 					<Parameter Name="Timeout">1000</Parameter>
      | 					<Parameter Name="BufferSize">50</Parameter>
      | 				</Parameters>
      | 			</SymbolControlItem>
      | 		</SymbolControlItems>
      | 	</Inputs>
      | 	<Outputs>
      | 		<SymbolControlItems>
      | 			<SymbolControlItem GroupName="ADS Read" GroupDescription="Parameters for ADS Read command">
      | 				<Parameters>
      | 					<Parameter Name="Name">MAIN.SchieberOben</Parameter>
      | 					<Parameter Name="SymbolName">MAIN.SchieberOben</Parameter>
      | 					<Parameter Name="SymbolType">BOOL</Parameter>
      | 					<Parameter Name="SymbolGuid">{18071995-0000-0000-0000-000000000030}</Parameter>
      | 					<Parameter Name="AmsNetId">192.168.8.155.1.1</Parameter>
      | 					<Parameter Name="Port">851</Parameter>
      | 					<Parameter Name="IndexGroup">#x0</Parameter>
      | 					<Parameter Name="IndexOffset">#x0</Parameter>
      | 					<Parameter Name="BitSize">8</Parameter>
      | 					<Parameter Name="InterpolationMode">3</Parameter>
      | 					<Parameter Name="ExtrapolationMode">0</Parameter>
      | 					<Parameter Name="SampleTime TC[100ns]">100000</Parameter>
      | 					<Parameter Name="SampleTime">100000</Parameter>
      | 					<Parameter Name="ReadViaNotification">True</Parameter>
      | 					<Parameter Name="Transmode">3</Parameter>
      | 					<Parameter Name="Timeout">1000</Parameter>
      | 					<Parameter Name="DelayTime">1000000</Parameter>
      | 					<Parameter Name="BufferSize">50</Parameter>
      | 				</Parameters>
      | 			</SymbolControlItem>
      | 		</SymbolControlItems>
      | 	</Outputs>
      | </PortInfo>
      settings: SourceProductName=Beckhoff TwinCAT Interface
  wires:
  Async ADS Read/1 -> NOT/1  "Busy"
  NOT/1 -> AND/1
  AND/1 -> Async ADS Read/1  "Trigger"
  Constant3/1 -> Async ADS Read/5  "IndexOffset"
  Constant2/1 -> Async ADS Read/4  "IndexGroup"
  Constant1/1 -> Async ADS Read/3  "Port"
  Constant/1 -> Async ADS Read/2  "NetId"
  Async ADS Read/2 -> Display/1  "Error"
  Async ADS Read/3 -> Display1/1  "Data"
  AND1/1 -> Async ADS Write/1  "Trigger"
  Square Wave Generator1/1 -> AND1/2
  NOT1/1 -> AND1/1
  Constant4/1 -> Async ADS Write/2  "NetId"
  Constant6/1 -> Async ADS Write/4  "IndexGroup"
  Constant5/1 -> Async ADS Write/3  "Port"
  Constant7/1 -> Async ADS Write/5  "IndexOffset"
  Constant8/1 -> Async ADS Write/6  "Data"
  Async ADS Write/2 -> Display3/1  "Error"
  Async ADS Write/1 -> Display2/1, NOT1/1  "Busy"
  FMU/1 -> Tc Symbol Interface/1, Display4/1  "MAIN.input1"
  FMU/2 -> Tc Symbol Interface/2, Display5/1  "MAIN.input2"
  FMU/3 -> Display6/1, Tc Symbol Interface/3  "MAIN.input3"
  Constant9/1 -> FMU/1
  Constant10/1 -> Cast To Boolean/1
  Cast To Boolean/1 -> FMU/2
  Constant12/1 -> FMU/5
  Tc Symbol Interface/1 -> Display7/1, Cast To Double/1  "MAIN.SchieberOben"
  Cast To Double/1 -> FMU/4
  Step/1 -> AND/2
